simulink model "kinovaMicoSimscapeModel"  (R2021b)
settings: Solver=VariableStepAuto  StartTime=0.0  StopTime=0.3  FixedStep=0.01  RelTol=1e-3
PostLoadFcn:
  | micoRigidBodyTreeCreation;
  | IC=deg2rad([-90,180,180,0,0,0]);
  | interactiveHomePosition=deg2rad([-90 90 177.5 90 0 0]');
  | load("./KinovaMicoSimscapeVariantConfigurations.mat");
values from neighbouring files (symbols this model uses):
  micoCandlePosition = deg2rad([0,180,180,0,0,0])    [KinovaMicoSimscapeInitializeScript.m]    (also in generatingRandomTrajectory.m)
  ViaPointsTaskSpace = [ViaPointsTaskSpace;[[pi;0;pi],[pi;0;pi],[pi;0;pi],[pi;0;pi],[0;0;0],[0;0;0],[pi;0;pi]]]    [KinovaMicoSimscapeInitializeScript.m]    (also in generatingRandomTrajectory.m = [ViaPointsTaskSpace;zeros(3,7)])
undefined symbols (not defined in the file or in its folder): Mico, ViaPointsJointSpace, X, Y, Z
libraries: sm_lib x26, nesl_utility x19, robotcorelib x4, robotmaniplib x3, pid_lib x2
(part 7 of 50)

== matlab function kinovaMicoSimscapeModel/Variant Subsystem/JointSpaceController/HybridImpedanceVelocityControl/C_RNE_SKEWSYMETRIC ==
  data: q input; C output; dq input
function C = fcn(q,dq)

%% Defining the position and velocity joint variables
q1 = q(1);
q2 = q(2);
q3 = q(3);
q4 = q(4);
q5 = q(5);
q6 = q(6);

dq1 = dq(1);
dq2 = dq(2);
dq3 = dq(3);
dq4 = dq(4);
dq5 = dq(5);
dq6 = dq(6);

%% Defining each entry in the matrix

C1_1 = 0.0009968*sin(q3 - 2.0*q2 + q4 + q5)*(dq3 - 2.0*dq2 + dq4 + dq5) - 0.0009968*sin(q3 + q4 + q5)*(dq3 + dq4 + dq5) + 0.0042912*sin(q3 + q4)*(dq3 + dq4) + 0.001151*sin(q3 + q5)*(dq3 + dq5) - 0.000096245*sin(q4 + q5)*(dq4 + dq5) + 0.074028*dq2*sin(2.0*q2) - 0.0010525*dq4*sin(2.0*q4) + 0.00016499*dq5*sin(2.0*q5) - 0.0042912*sin(q3 - 2.0*q2 + q4)*(dq3 - 2.0*dq2 + dq4) - 0.001151*sin(q3 - 2.0*q2 + q5)*(dq3 - 2.0*dq2 + dq5) + 0.00033227*sin(q3 + q4 - 1.0*q5)*(dq3 + dq4 - 1.0*dq5) - 0.00033227*sin(q3 - 1.0*q4 + q5)*(dq3 - 1.0*dq4 + dq5) + 0.0009968*sin(q4 - 1.0*q3 + q5)*(dq4 - 1.0*dq3 + dq5) - 0.0009968*sin(2.0*q2 - 1.0*q3 + q4 + q5)*(2.0*dq2 - 1.0*dq3 + dq4 + dq5) - 0.00057005*sin(2.0*q3 - 2.0*q2 + q4 + q5)*(2.0*dq3 - 2.0*dq2 + dq4 + dq5) + 0.00057005*sin(2.0*q2 - 2.0*q3 + q4 + q5)*(2.0*dq2 - 2.0*dq3 + dq4 + dq5) - 0.0042912*sin(q3 - 1.0*q4)*(dq3 - 1.0*dq4) + 0.001151*sin(q3 - 1.0*q5)*(dq3 - 1.0*dq5) + 0.000032082*sin(q4 - 1.0*q5)*(dq4 - 1.0*dq5) + 0.00009067*sin(2.0*q4 + q5)*(2.0*dq4 + dq5) + 0.0042912*sin(2.0*q2 - 1.0*q3 + q4)*(2.0*dq2 - 1.0*dq3 + dq4) + 0.0025555*sin(2.0*q3 - 2.0*q2 + q4)*(2.0*dq3 - 2.0*dq2 + dq4) - 0.001151*sin(2.0*q2 - 1.0*q3 + q5)*(2.0*dq2 - 1.0*dq3 + dq5) - 0.0025555*sin(2.0*q2 - 2.0*q3 + q4)*(2.0*dq2 - 2.0*dq3 + dq4) + 0.0007489*sin(2.0*q3 - 2.0*q2 + q5)*(2.0*dq3 - 2.0*dq2 + dq5) + 0.0007489*sin(2.0*q2 - 2.0*q3 + q5)*(2.0*dq2 - 2.0*dq3 + dq5) + 0.00033227*sin(2.0*q2 - 1.0*q3 + q4 - 1.0*q5)*(2.0*dq2 - 1.0*dq3 + dq4 - 1.0*dq5) - 0.00033227*sin(2.0*q2 - 1.0*q3 - 1.0*q4 + q5)*(2.0*dq2 - 1.0*dq3 - 1.0*dq4 + dq5) - 0.00025981*sin(2.0*q2 - 2.0*q3 + q4 - 1.0*q5)*(2.0*dq2 - 2.0*dq3 + dq4 - 1.0*dq5) + 0.00025981*sin(2.0*q2 - 2.0*q3 - 1.0*q4 + q5)*(2.0*dq2 - 2.0*dq3 - 1.0*dq4 + dq5) - 0.00014289*sin(2.0*q3 - 2.0*q2 + q4 + 2.0*q5)*(2.0*dq3 - 2.0*dq2 + dq4 + 2.0*dq5) - 0.000045334*sin(2.0*q3 - 2.0*q2 + 2.0*q4 + q5)*(2.0*dq3 - 2.0*dq2 + 2.0*dq4 + dq5) - 0.000047629*sin(2.0*q2 - 2.0*q3 + q4 - 2.0*q5)*(2.0*dq2 - 2.0*dq3 + dq4 - 2.0*dq5) + 0.00014289*sin(2.0*q2 - 2.0*q3 + q4 + 2.0*q5)*(2.0*dq2 - 2.0*dq3 + dq4 + 2.0*dq5) + 0.000015111*sin(2.0*q2 - 2.0*q3 - 2.0*q4 + q5)*(2.0*dq2 - 2.0*dq3 - 2.0*dq4 + dq5) - 0.000045334*sin(2.0*q2 - 2.0*q3 + 2.0*q4 + q5)*(2.0*dq2 - 2.0*dq3 + 2.0*dq4 + dq5) + 0.030397*dq3*sin(q3) + 0.00041432*dq4*sin(q4) - 0.001256*dq5*sin(q5) - 0.030397*sin(2.0*q2 - 1.0*q3)*(2.0*dq2 - 1.0*dq3) + 0.009146*sin(2.0*q2 - 2.0*q3)*(2.0*dq2 - 2.0*dq3) - 0.000030222*sin(2.0*q4 - 1.0*q5)*(2.0*dq4 - 1.0*dq5) - 0.000013749*sin(2.0*q4 - 2.0*q5)*(2.0*dq4 - 2.0*dq5) - 0.00012375*sin(2.0*q4 + 2.0*q5)*(2.0*dq4 + 2.0*dq5) + 0.00026314*sin(2.0*q3 - 2.0*q2 + 2.0*q4)*(2.0*dq3 - 2.0*dq2 + 2.0*dq4) + 0.00026314*sin(2.0*q2 - 2.0*q3 + 2.0*q4)*(2.0*dq2 - 2.0*dq3 + 2.0*dq4) + 0.00012375*sin(2.0*q3 - 2.0*q2 + 2.0*q5)*(2.0*dq3 - 2.0*dq2 + 2.0*dq5) + 0.00012375*sin(2.0*q2 - 2.0*q3 + 2.0*q5)*(2.0*dq2 - 2.0*dq3 + 2.0*dq5) + 0.000047629*sin(2.0*q2 - 2.0*q3 - 1.0*q4 + 2.0*q5)*(2.0*dq2 - 2.0*dq3 - 1.0*dq4 + 2.0*dq5) + 0.000015111*sin(2.0*q2 - 2.0*q3 + 2.0*q4 - 1.0*q5)*(2.0*dq2 - 2.0*dq3 + 2.0*dq4 - 1.0*dq5) + 0.00006187*sin(2.0*q3 - 2.0*q2 + 2.0*q4 + 2.0*q5)*(2.0*dq3 - 2.0*dq2 + 2.0*dq4 + 2.0*dq5) + 6.8745e-6*sin(2.0*q2 - 2.0*q3 - 2.0*q4 + 2.0*q5)*(2.0*dq2 - 2.0*dq3 - 2.0*dq4 + 2.0*dq5) + 6.8745e-6*sin(2.0*q2 - 2.0*q3 + 2.0*q4 - 2.0*q5)*(2.0*dq2 - 2.0*dq3 + 2.0*dq4 - 2.0*dq5) + 0.00006187*sin(2.0*q2 - 2.0*q3 + 2.0*q4 + 2.0*q5)*(2.0*dq2 - 2.0*dq3 + 2.0*dq4 + 2.0*dq5);
 
C1_2 = 0.074028*dq1*sin(2.0*q2) + 0.0034131*dq2*sin(q2) + 0.060795*dq1*cos(2.0*q2)*sin(q3) - 0.060795*dq1*sin(2.0*q2)*cos(q3) + 0.0010437*dq2*cos(q2)*sin(q3) - 0.0010437*dq2*cos(q3)*sin(q2) - 0.017165*dq2*cos(q4)*sin(q2) - 0.0010437*dq3*cos(q2)*sin(q3) + 0.0010437*dq3*cos(q3)*sin(q2) + 0.0034398*dq4*cos(q2)*sin(q3) - 0.0034398*dq4*cos(q3)*sin(q2) + 0.0006317*dq5*cos(q2)*sin(q3) - 0.0006317*dq5*cos(q3)*sin(q2) + 0.000078*dq6*cos(q2)*sin(q3) - 0.000078*dq6*cos(q3)*sin(q2) - 0.018292*dq1*cos(2.0*q2)*sin(2.0*q3) + 0.018292*dq1*cos(2.0*q3)*sin(2.0*q2) + 0.017165*dq1*sin(2.0*q2)*sin(q3)*sin(q4) - 0.002105*dq2*sin(2.0*q4)*sin(q2)*sin(q3) + 0.002105*dq3*sin(2.0*q4)*sin(q2)*sin(q3) - 0.0010525*dq1*cos(2.0*q2)*cos(2.0*q4)*sin(2.0*q3) + 0.0010525*dq1*cos(2.0*q3)*cos(2.0*q4)*sin(2.0*q2) - 0.00049498*dq1*cos(2.0*q2)*cos(2.0*q5)*sin(2.0*q3) + 0.00049498*dq1*cos(2.0*q3)*cos(2.0*q5)*sin(2.0*q2) + 0.0004144*dq2*cos(q2)*cos(q3)*sin(q4) - 0.010222*dq2*cos(q2)*cos(q4)*sin(q3) + 0.010222*dq2*cos(q3)*cos(q4)*sin(q2) + 0.00011113*dq2*cos(q2)*cos(q5)*sin(q3) - 0.00011113*dq2*cos(q3)*cos(q5)*sin(q2) - 0.0004144*dq3*cos(q2)*cos(q3)*sin(q4) + 0.010222*dq3*cos(q2)*cos(q4)*sin(q3) - 0.010222*dq3*cos(q3)*cos(q4)*sin(q2) + 0.0026581*dq2*cos(q4)*cos(q5)*sin(q2) - 0.00011113*dq3*cos(q2)*cos(q5)*sin(q3) + 0.00011113*dq3*cos(q3)*cos(q5)*sin(q2) - 0.0004144*dq4*cos(q2)*cos(q4)*sin(q3) + 0.0004144*dq4*cos(q3)*cos(q4)*sin(q2) - 0.00024178*dq4*cos(q2)*cos(q5)*sin(q3) + 0.00024178*dq4*cos(q3)*cos(q5)*sin(q2) + 0.0010941*dq5*cos(q2)*cos(q3)*sin(q4) - 0.00011114*dq5*cos(q2)*cos(q3)*sin(q5) - 0.00024178*dq5*cos(q2)*cos(q5)*sin(q3) + 0.00024178*dq5*cos(q3)*cos(q5)*sin(q2) + 0.0001351*dq6*cos(q2)*cos(q3)*sin(q4) + 0.000234*dq6*cos(q2)*cos(q5)*sin(q3) - 0.000234*dq6*cos(q3)*cos(q5)*sin(q2) + 0.0004144*dq2*sin(q2)*sin(q3)*sin(q4) - 0.0004144*dq3*sin(q2)*sin(q3)*sin(q4) - 0.0053163*dq2*sin(q2)*sin(q4)*sin(q5) + 0.0010941*dq5*sin(q2)*sin(q3)*sin(q4) - 0.00011114*dq5*sin(q2)*sin(q3)*sin(q5) + 0.0001351*dq6*sin(q2)*sin(q3)*sin(q4) - 0.010222*dq1*cos(2.0*q2)*cos(2.0*q3)*sin(q4) - 0.0029956*dq1*cos(2.0*q2)*sin(2.0*q3)*cos(q5) + 0.0029956*dq1*cos(2.0*q3)*sin(2.0*q2)*cos(q5) - 0.010222*dq1*sin(2.0*q2)*sin(2.0*q3)*sin(q4) + 0.017165*dq1*cos(2.0*q2)*cos(q3)*sin(q4) + 0.004604*dq1*cos(2.0*q2)*cos(q5)*sin(q3) - 0.004604*dq1*sin(2.0*q2)*cos(q3)*cos(q5) - 0.002105*dq2*sin(2.0*q4)*cos(q2)*cos(q3) + 0.002105*dq3*sin(2.0*q4)*cos(q2)*cos(q3) + 0.002105*dq4*cos(2.0*q4)*cos(q2)*sin(q3) - 0.002105*dq4*cos(2.0*q4)*cos(q3)*sin(q2) - 0.00032998*dq4*cos(2.0*q5)*cos(q2)*sin(q3) + 0.00032998*dq4*cos(2.0*q5)*cos(q3)*sin(q2) + 0.00038102*dq1*cos(2.0*q2)*cos(2.0*q3)*cos(2.0*q5)*sin(q4) + 0.00076206*dq1*cos(2.0*q2)*cos(2.0*q3)*sin(2.0*q5)*cos(q4) + 0.00012089*dq1*cos(2.0*q2)*cos(2.0*q4)*sin(2.0*q3)*cos(q5) - 0.00012089*dq1*cos(2.0*q3)*cos(2.0*q4)*sin(2.0*q2)*cos(q5) - 0.00024178*dq1*cos(2.0*q2)*sin(2.0*q3)*sin(2.0*q4)*sin(q5) + 0.00024178*dq1*cos(2.0*q3)*sin(2.0*q2)*sin(2.0*q4)*sin(q5) + 0.00038102*dq1*cos(2.0*q5)*sin(2.0*q2)*sin(2.0*q3)*sin(q4) + 0.00076206*dq1*sin(2.0*q2)*sin(2.0*q3)*sin(2.0*q5)*cos(q4) - 0.00012839*dq2*cos(q2)*cos(q3)*cos(q4)*sin(q5) - 0.00006421*dq2*cos(q2)*cos(q3)*cos(q5)*sin(q4) + 0.0012409*dq2*cos(q2)*cos(q4)*cos(q5)*sin(q3) - 0.0012409*dq2*cos(q3)*cos(q4)*cos(q5)*sin(q2) + 0.00012839*dq3*cos(q2)*cos(q3)*cos(q4)*sin(q5) + 0.00006421*dq3*cos(q2)*cos(q3)*cos(q5)*sin(q4) - 0.0012409*dq3*cos(q2)*cos(q4)*cos(q5)*sin(q3) + 0.0012409*dq3*cos(q3)*cos(q4)*cos(q5)*sin(q2) + 0.00006421*dq4*cos(q2)*cos(q4)*cos(q5)*sin(q3) - 0.00006421*dq4*cos(q3)*cos(q4)*cos(q5)*sin(q2) + 0.00041878*dq5*cos(q2)*cos(q3)*cos(q4)*sin(q5) + 1.5e-8*dq5*cos(q2)*cos(q3)*cos(q5)*sin(q4) + 0.00012839*dq5*cos(q2)*cos(q4)*cos(q5)*sin(q3) - 0.00012839*dq5*cos(q3)*cos(q4)*cos(q5)*sin(q2) - 0.0002702*dq6*cos(q2)*cos(q3)*cos(q4)*sin(q5) - 0.0001351*dq6*cos(q2)*cos(q3)*cos(q5)*sin(q4) - 0.0033193*dq2*cos(q2)*sin(q3)*sin(q4)*sin(q5) + 0.0033193*dq2*cos(q3)*sin(q2)*sin(q4)*sin(q5) - 0.00012839*dq2*cos(q4)*sin(q2)*sin(q3)*sin(q5) - 0.00006421*dq2*cos(q5)*sin(q2)*sin(q3)*sin(q4) + 0.0033193*dq3*cos(q2)*sin(q3)*sin(q4)*sin(q5) - 0.0033193*dq3*cos(q3)*sin(q2)*sin(q4)*sin(q5) + 0.00012839*dq3*cos(q4)*sin(q2)*sin(q3)*sin(q5) + 0.00006421*dq3*cos(q5)*sin(q2)*sin(q3)*sin(q4) - 0.00012839*dq4*cos(q2)*sin(q3)*sin(q4)*sin(q5) + 0.00012839*dq4*cos(q3)*sin(q2)*sin(q4)*sin(q5) - 0.000064215*dq5*cos(q2)*sin(q3)*sin(q4)*sin(q5) + 0.000064215*dq5*cos(q3)*sin(q2)*sin(q4)*sin(q5) + 0.00041878*dq5*cos(q4)*sin(q2)*sin(q3)*sin(q5) + 1.5e-8*dq5*cos(q5)*sin(q2)*sin(q3)*sin(q4) - 0.0002702*dq6*cos(q4)*sin(q2)*sin(q3)*sin(q5) - 0.0001351*dq6*cos(q5)*sin(q2)*sin(q3)*sin(q4) + 0.0033194*dq1*cos(2.0*q2)*cos(2.0*q3)*cos(q4)*sin(q5) + 0.001241*dq1*cos(2.0*q2)*cos(2.0*q3)*cos(q5)*sin(q4) - 0.00043998*dq2*cos(2.0*q4)*sin(2.0*q5)*cos(q2)*cos(q3) - 0.00054998*dq2*cos(2.0*q5)*sin(2.0*q4)*cos(q2)*cos(q3) + 0.00043998*dq3*cos(2.0*q4)*sin(2.0*q5)*cos(q2)*cos(q3) + 0.00054998*dq3*cos(2.0*q5)*sin(2.0*q4)*cos(q2)*cos(q3) + 0.00054998*dq4*cos(2.0*q4)*cos(2.0*q5)*cos(q2)*sin(q3) - 0.00054998*dq4*cos(2.0*q4)*cos(2.0*q5)*cos(q3)*sin(q2) + 0.00043998*dq5*cos(2.0*q4)*cos(2.0*q5)*cos(q2)*sin(q3) - 0.00043998*dq5*cos(2.0*q4)*cos(2.0*q5)*cos(q3)*sin(q2) + 0.0033194*dq1*sin(2.0*q2)*sin(2.0*q3)*cos(q4)*sin(q5) + 0.001241*dq1*sin(2.0*q2)*sin(2.0*q3)*cos(q5)*sin(q4) - 0.00043998*dq2*cos(2.0*q4)*sin(2.0*q5)*sin(q2)*sin(q3) - 0.00054998*dq2*cos(2.0*q5)*sin(2.0*q4)*sin(q2)*sin(q3) + 0.00043998*dq3*cos(2.0*q4)*sin(2.0*q5)*sin(q2)*sin(q3) + 0.00054998*dq3*cos(2.0*q5)*sin(2.0*q4)*sin(q2)*sin(q3) - 0.00043998*dq4*sin(2.0*q4)*sin(2.0*q5)*cos(q2)*sin(q3) + 0.00043998*dq4*sin(2.0*q4)*sin(2.0*q5)*cos(q3)*sin(q2) - 0.00054998*dq5*sin(2.0*q4)*sin(2.0*q5)*cos(q2)*sin(q3) + 0.00054998*dq5*sin(2.0*q4)*sin(2.0*q5)*cos(q3)*sin(q2) - 0.00027498*dq1*cos(2.0*q2)*cos(2.0*q4)*cos(2.0*q5)*sin(2.0*q3) + 0.00027498*dq1*cos(2.0*q3)*cos(2.0*q4)*cos(2.0*q5)*sin(2.0*q2) + 0.00021998*dq1*cos(2.0*q2)*sin(2.0*q3)*sin(2.0*q4)*sin(2.0*q5) - 0.00021998*dq1*cos(2.0*q3)*sin(2.0*q2)*sin(2.0*q4)*sin(2.0*q5) - 0.0053163*dq1*cos(2.0*q2)*cos(q3)*cos(q4)*sin(q5) - 0.0026581*dq1*cos(2.0*q2)*cos(q3)*cos(q5)*sin(q4) + 0.00048357*dq2*cos(2.0*q4)*cos(q2)*cos(q3)*sin(q5) + 0.00038102*dq2*cos(2.0*q5)*cos(q2)*cos(q4)*sin(q3) - 0.00038102*dq2*cos(2.0*q5)*cos(q3)*cos(q4)*sin(q2) + 0.00024179*dq2*sin(2.0*q4)*cos(q2)*cos(q3)*cos(q5) - 0.00048357*dq3*cos(2.0*q4)*cos(q2)*cos(q3)*sin(q5) - 0.00038102*dq3*cos(2.0*q5)*cos(q2)*cos(q4)*sin(q3) + 0.00038102*dq3*cos(2.0*q5)*cos(q3)*cos(q4)*sin(q2) - 0.00024179*dq3*sin(2.0*q4)*cos(q2)*cos(q3)*cos(q5) - 0.00024179*dq4*cos(2.0*q4)*cos(q2)*cos(q5)*sin(q3) + 0.00024179*dq4*cos(2.0*q4)*cos(q3)*cos(q5)*sin(q2) - 0.00024178*dq5*cos(2.0*q4)*cos(q2)*cos(q5)*sin(q3) + 0.00024178*dq5*cos(2.0*q4)*cos(q3)*cos(q5)*sin(q2) - 0.00076206*dq5*cos(2.0*q5)*cos(q2)*cos(q3)*sin(q4) - 0.00038102*dq5*sin(2.0*q5)*cos(q2)*cos(q3)*cos(q4) - 0.0053163*dq1*sin(2.0*q2)*cos(q4)*sin(q3)*sin(q5) - 0.0026581*dq1*sin(2.0*q2)*cos(q5)*sin(q3)*sin(q4) + 0.00048357*dq2*cos(2.0*q4)*sin(q2)*sin(q3)*sin(q5) + 0.00024179*dq2*sin(2.0*q4)*cos(q5)*sin(q2)*sin(q3) - 0.00076206*dq2*sin(2.0*q5)*cos(q2)*sin(q3)*sin(q4) + 0.00076206*dq2*sin(2.0*q5)*cos(q3)*sin(q2)*sin(q4) - 0.00048357*dq3*cos(2.0*q4)*sin(q2)*sin(q3)*sin(q5) - 0.00024179*dq3*sin(2.0*q4)*cos(q5)*sin(q2)*sin(q3) + 0.00076206*dq3*sin(2.0*q5)*cos(q2)*sin(q3)*sin(q4) - 0.00076206*dq3*sin(2.0*q5)*cos(q3)*sin(q2)*sin(q4) + 0.00048357*dq4*sin(2.0*q4)*cos(q2)*sin(q3)*sin(q5) - 0.00048357*dq4*sin(2.0*q4)*cos(q3)*sin(q2)*sin(q5) - 0.00076206*dq5*cos(2.0*q5)*sin(q2)*sin(q3)*sin(q4) + 0.00012089*dq5*sin(2.0*q4)*cos(q2)*sin(q3)*sin(q5) - 0.00012089*dq5*sin(2.0*q4)*cos(q3)*sin(q2)*sin(q5) - 0.00038102*dq5*sin(2.0*q5)*cos(q4)*sin(q2)*sin(q3);
 
C1_3 = 0.030397*dq1*sin(q3) - 0.030397*dq1*cos(2.0*q2)*sin(q3) + 0.030397*dq1*sin(2.0*q2)*cos(q3) - 0.0010437*dq2*cos(q2)*sin(q3) + 0.0010437*dq2*cos(q3)*sin(q2) + 0.0085823*dq1*cos(q3)*sin(q4) + 0.0010437*dq3*cos(q2)*sin(q3) - 0.0010437*dq3*cos(q3)*sin(q2) + 0.002302*dq1*cos(q5)*sin(q3) - 0.0034398*dq4*cos(q2)*sin(q3) + 0.0034398*dq4*cos(q3)*sin(q2) - 0.0006317*dq5*cos(q2)*sin(q3) + 0.0006317*dq5*cos(q3)*sin(q2) - 0.000078*dq6*cos(q2)*sin(q3) + 0.000078*dq6*cos(q3)*sin(q2) + 0.018292*dq1*cos(2.0*q2)*sin(2.0*q3) - 0.018292*dq1*cos(2.0*q3)*sin(2.0*q2) - 0.0085823*dq1*sin(2.0*q2)*sin(q3)*sin(q4) + 0.002105*dq2*sin(2.0*q4)*sin(q2)*sin(q3) - 0.002105*dq3*sin(2.0*q4)*sin(q2)*sin(q3) + 0.0010525*dq1*cos(2.0*q2)*cos(2.0*q4)*sin(2.0*q3) - 0.0010525*dq1*cos(2.0*q3)*cos(2.0*q4)*sin(2.0*q2) + 0.00049498*dq1*cos(2.0*q2)*cos(2.0*q5)*sin(2.0*q3) - 0.00049498*dq1*cos(2.0*q3)*cos(2.0*q5)*sin(2.0*q2) - 0.0004144*dq2*cos(q2)*cos(q3)*sin(q4) + 0.010222*dq2*cos(q2)*cos(q4)*sin(q3) - 0.010222*dq2*cos(q3)*cos(q4)*sin(q2) - 0.00011113*dq2*cos(q2)*cos(q5)*sin(q3) + 0.00011113*dq2*cos(q3)*cos(q5)*sin(q2) + 0.0004144*dq3*cos(q2)*cos(q3)*sin(q4) - 0.010222*dq3*cos(q2)*cos(q4)*sin(q3) + 0.010222*dq3*cos(q3)*cos(q4)*sin(q2) - 0.0026581*dq1*cos(q3)*cos(q4)*sin(q5) - 0.0013291*dq1*cos(q3)*cos(q5)*sin(q4) + 0.00011113*dq3*cos(q2)*cos(q5)*sin(q3) - 0.00011113*dq3*cos(q3)*cos(q5)*sin(q2) + 0.0004144*dq4*cos(q2)*cos(q4)*sin(q3) - 0.0004144*dq4*cos(q3)*cos(q4)*sin(q2) + 0.00024178*dq4*cos(q2)*cos(q5)*sin(q3) - 0.00024178*dq4*cos(q3)*cos(q5)*sin(q2) - 0.0010941*dq5*cos(q2)*cos(q3)*sin(q4) + 0.00011114*dq5*cos(q2)*cos(q3)*sin(q5) + 0.00024178*dq5*cos(q2)*cos(q5)*sin(q3) - 0.00024178*dq5*cos(q3)*cos(q5)*sin(q2) - 0.0001351*dq6*cos(q2)*cos(q3)*sin(q4) - 0.000234*dq6*cos(q2)*cos(q5)*sin(q3) + 0.000234*dq6*cos(q3)*cos(q5)*sin(q2) - 0.0004144*dq2*sin(q2)*sin(q3)*sin(q4) + 0.0004144*dq3*sin(q2)*sin(q3)*sin(q4) - 0.0010941*dq5*sin(q2)*sin(q3)*sin(q4) + 0.00011114*dq5*sin(q2)*sin(q3)*sin(q5) - 0.0001351*dq6*sin(q2)*sin(q3)*sin(q4) + 0.010222*dq1*cos(2.0*q2)*cos(2.0*q3)*sin(q4) + 0.0029956*dq1*cos(2.0*q2)*sin(2.0*q3)*cos(q5) - 0.0029956*dq1*cos(2.0*q3)*sin(2.0*q2)*cos(q5) + 0.010222*dq1*sin(2.0*q2)*sin(2.0*q3)*sin(q4) - 0.0085823*dq1*cos(2.0*q2)*cos(q3)*sin(q4) - 0.002302*dq1*cos(2.0*q2)*cos(q5)*sin(q3) + 0.002302*dq1*sin(2.0*q2)*cos(q3)*cos(q5) + 0.002105*dq2*sin(2.0*q4)*cos(q2)*cos(q3) - 0.002105*dq3*sin(2.0*q4)*cos(q2)*cos(q3) - 0.002105*dq4*cos(2.0*q4)*cos(q2)*sin(q3) + 0.002105*dq4*cos(2.0*q4)*cos(q3)*sin(q2) + 0.00032998*dq4*cos(2.0*q5)*cos(q2)*sin(q3) - 0.00032998*dq4*cos(2.0*q5)*cos(q3)*sin(q2) - 0.00038102*dq1*cos(2.0*q2)*cos(2.0*q3)*cos(2.0*q5)*sin(q4) - 0.00076206*dq1*cos(2.0*q2)*cos(2.0*q3)*sin(2.0*q5)*cos(q4) - 0.00012089*dq1*cos(2.0*q2)*cos(2.0*q4)*sin(2.0*q3)*cos(q5) + 0.00012089*dq1*cos(2.0*q3)*cos(2.0*q4)*sin(2.0*q2)*cos(q5) + 0.00024178*dq1*cos(2.0*q2)*sin(2.0*q3)*sin(2.0*q4)*sin(q5) - 0.00024178*dq1*cos(2.0*q3)*sin(2.0*q2)*sin(2.0*q4)*sin(q5) - 0.00038102*dq1*cos(2.0*q5)*sin(2.0*q2)*sin(2.0*q3)*sin(q4) - 0.00076206*dq1*sin(2.0*q2)*sin(2.0*q3)*sin(2.0*q5)*cos(q4) + 0.00012839*dq2*cos(q2)*cos(q3)*cos(q4)*sin(q5) + 0.00006421*dq2*cos(q2)*cos(q3)*cos(q5)*sin(q4) - 0.0012409*dq2*cos(q2)*cos(q4)*cos(q5)*sin(q3) + 0.0012409*dq2*cos(q3)*cos(q4)*cos(q5)*sin(q2) - 0.00012839*dq3*cos(q2)*cos(q3)*cos(q4)*sin(q5) - 0.00006421*dq3*cos(q2)*cos(q3)*cos(q5)*sin(q4) + 0.0012409*dq3*cos(q2)*cos(q4)*cos(q5)*sin(q3) - 0.0012409*dq3*cos(q3)*cos(q4)*cos(q5)*sin(q2) - 0.00006421*dq4*cos(q2)*cos(q4)*cos(q5)*sin(q3) + 0.00006421*dq4*cos(q3)*cos(q4)*cos(q5)*sin(q2) - 0.00041878*dq5*cos(q2)*cos(q3)*cos(q4)*sin(q5) - 1.5e-8*dq5*cos(q2)*cos(q3)*cos(q5)*sin(q4) - 0.00012839*dq5*cos(q2)*cos(q4)*cos(q5)*sin(q3) + 0.00012839*dq5*cos(q3)*cos(q4)*cos(q5)*sin(q2) + 0.0002702*dq6*cos(q2)*cos(q3)*cos(q4)*sin(q5) + 0.0001351*dq6*cos(q2)*cos(q3)*cos(q5)*sin(q4) + 0.0033193*dq2*cos(q2)*sin(q3)*sin(q4)*sin(q5) - 0.0033193*dq2*cos(q3)*sin(q2)*sin(q4)*sin(q5) + 0.00012839*dq2*cos(q4)*sin(q2)*sin(q3)*sin(q5) + 0.00006421*dq2*cos(q5)*sin(q2)*sin(q3)*sin(q4) - 0.0033193*dq3*cos(q2)*sin(q3)*sin(q4)*sin(q5) + 0.0033193*dq3*cos(q3)*sin(q2)*sin(q4)*sin(q5) - 0.00012839*dq3*cos(q4)*sin(q2)*sin(q3)*sin(q5) - 0.00006421*dq3*cos(q5)*sin(q2)*sin(q3)*sin(q4) + 0.00012839*dq4*cos(q2)*sin(q3)*sin(q4)*sin(q5) - 0.00012839*dq4*cos(q3)*sin(q2)*sin(q4)*sin(q5) + 0.000064215*dq5*cos(q2)*sin(q3)*sin(q4)*sin(q5) - 0.000064215*dq5*cos(q3)*sin(q2)*sin(q4)*sin(q5) - 0.00041878*dq5*cos(q4)*sin(q2)*sin(q3)*sin(q5) - 1.5e-8*dq5*cos(q5)*sin(q2)*sin(q3)*sin(q4) + 0.0002702*dq6*cos(q4)*sin(q2)*sin(q3)*sin(q5) + 0.0001351*dq6*cos(q5)*sin(q2)*sin(q3)*sin(q4) - 0.0033194*dq1*cos(2.0*q2)*cos(2.0*q3)*cos(q4)*sin(q5) - 0.001241*dq1*cos(2.0*q2)*cos(2.0*q3)*cos(q5)*sin(q4) + 0.00043998*dq2*cos(2.0*q4)*sin(2.0*q5)*cos(q2)*cos(q3) + 0.00054998*dq2*cos(2.0*q5)*sin(2.0*q4)*cos(q2)*cos(q3) - 0.00043998*dq3*cos(2.0*q4)*sin(2.0*q5)*cos(q2)*cos(q3) - 0.00054998*dq3*cos(2.0*q5)*sin(2.0*q4)*cos(q2)*cos(q3) - 0.00054998*dq4*cos(2.0*q4)*cos(2.0*q5)*cos(q2)*sin(q3) + 0.00054998*dq4*cos(2.0*q4)*cos(2.0*q5)*cos(q3)*sin(q2) - 0.00043998*dq5*cos(2.0*q4)*cos(2.0*q5)*cos(q2)*sin(q3) + 0.00043998*dq5*cos(2.0*q4)*cos(2.0*q5)*cos(q3)*sin(q2) - 0.0033194*dq1*sin(2.0*q2)*sin(2.0*q3)*cos(q4)*sin(q5) - 0.001241*dq1*sin(2.0*q2)*sin(2.0*q3)*cos(q5)*sin(q4) + 0.00043998*dq2*cos(2.0*q4)*sin(2.0*q5)*sin(q2)*sin(q3) + 0.00054998*dq2*cos(2.0*q5)*sin(2.0*q4)*sin(q2)*sin(q3) - 0.00043998*dq3*cos(2.0*q4)*sin(2.0*q5)*sin(q2)*sin(q3) - 0.00054998*dq3*cos(2.0*q5)*sin(2.0*q4)*sin(q2)*sin(q3) + 0.00043998*dq4*sin(2.0*q4)*sin(2.0*q5)*cos(q2)*sin(q3) - 0.00043998*dq4*sin(2.0*q4)*sin(2.0*q5)*cos(q3)*sin(q2) + 0.00054998*dq5*sin(2.0*q4)*sin(2.0*q5)*cos(q2)*sin(q3) - 0.00054998*dq5*sin(2.0*q4)*sin(2.0*q5)*cos(q3)*sin(q2) + 0.00027498*dq1*cos(2.0*q2)*cos(2.0*q4)*cos(2.0*q5)*sin(2.0*q3) - 0.00027498*dq1*cos(2.0*q3)*cos(2.0*q4)*cos(2.0*q5)*sin(2.0*q2) - 0.00021998*dq1*cos(2.0*q2)*sin(2.0*q3)*sin(2.0*q4)*sin(2.0*q5) + 0.00021998*dq1*cos(2.0*q3)*sin(2.0*q2)*sin(2.0*q4)*sin(2.0*q5) + 0.0026581*dq1*cos(2.0*q2)*cos(q3)*cos(q4)*sin(q5) + 0.0013291*dq1*cos(2.0*q2)*cos(q3)*cos(q5)*sin(q4) - 0.00048357*dq2*cos(2.0*q4)*cos(q2)*cos(q3)*sin(q5) - 0.00038102*dq2*cos(2.0*q5)*cos(q2)*cos(q4)*sin(q3) + 0.00038102*dq2*cos(2.0*q5)*cos(q3)*cos(q4)*sin(q2) - 0.00024179*dq2*sin(2.0*q4)*cos(q2)*cos(q3)*cos(q5) + 0.00048357*dq3*cos(2.0*q4)*cos(q2)*cos(q3)*sin(q5) + 0.00038102*dq3*cos(2.0*q5)*cos(q2)*cos(q4)*sin(q3) - 0.00038102*dq3*cos(2.0*q5)*cos(q3)*cos(q4)*sin(q2) + 0.00024179*dq3*sin(2.0*q4)*cos(q2)*cos(q3)*cos(q5) + 0.00024179*dq4*cos(2.0*q4)*cos(q2)*cos(q5)*sin(q3) - 0.00024179*dq4*cos(2.0*q4)*cos(q3)*cos(q5)*sin(q2) + 0.00024178*dq5*cos(2.0*q4)*cos(q2)*cos(q5)*sin(q3) - 0.00024178*dq5*cos(2.0*q4)*cos(q3)*cos(q5)*sin(q2) + 0.00076206*dq5*cos(2.0*q5)*cos(q2)*cos(q3)*sin(q4) + 0.00038102*dq5*sin(2.0*q5)*cos(q2)*cos(q3)*cos(q4) + 0.0026581*dq1*sin(2.0*q2)*cos(q4)*sin(q3)*sin(q5) + 0.0013291*dq1*sin(2.0*q2)*cos(q5)*sin(q3)*sin(q4) - 0.00048357*dq2*cos(2.0*q4)*sin(q2)*sin(q3)*sin(q5) - 0.00024179*dq2*sin(2.0*q4)*cos(q5)*sin(q2)*sin(q3) + 0.00076206*dq2*sin(2.0*q5)*cos(q2)*sin(q3)*sin(q4) - 0.00076206*dq2*sin(2.0*q5)*cos(q3)*sin(q2)*sin(q4) + 0.00048357*dq3*cos(2.0*q4)*sin(q2)*sin(q3)*sin(q5) + 0.00024179*dq3*sin(2.0*q4)*cos(q5)*sin(q2)*sin(q3) - 0.00076206*dq3*sin(2.0*q5)*cos(q2)*sin(q3)*sin(q4) + 0.00076206*dq3*sin(2.0*q5)*cos(q3)*sin(q2)*sin(q4) - 0.00048357*dq4*sin(2.0*q4)*cos(q2)*sin(q3)*sin(q5) + 0.00048357*dq4*sin(2.0*q4)*cos(q3)*sin(q2)*sin(q5) + 0.00076206*dq5*cos(2.0*q5)*sin(q2)*sin(q3)*sin(q4) - 0.00012089*dq5*sin(2.0*q4)*cos(q2)*sin(q3)*sin(q5) + 0.00012089*dq5*sin(2.0*q4)*cos(q3)*sin(q2)*sin(q5) + 0.00038102*dq5*sin(2.0*q5)*cos(q4)*sin(q2)*sin(q3);
 
C1_4 = 0.00041432*dq1*sin(q4) - 0.0010525*dq1*sin(2.0*q4) + 0.00024178*dq1*cos(2.0*q4)*sin(q5) + 0.00012089*dq1*sin(2.0*q4)*cos(q5) + 0.0034398*dq2*cos(q2)*sin(q3) - 0.0034398*dq2*cos(q3)*sin(q2) + 0.0085823*dq1*cos(q4)*sin(q3) - 0.0034398*dq3*cos(q2)*sin(q3) + 0.0034398*dq3*cos(q3)*sin(q2) - 0.00012833*dq1*cos(q4)*sin(q5) - 0.000064164*dq1*cos(q5)*sin(q4) + 0.017165*dq4*cos(q4)*sin(q2) - 0.00021999*dq1*cos(2.0*q4)*sin(2.0*q5) - 0.00027499*dq1*cos(2.0*q5)*sin(2.0*q4) + 0.00065996*dq5*sin(2.0*q5)*sin(q2)*sin(q3) + 0.0010525*dq1*cos(2.0*q2)*cos(2.0*q3)*sin(2.0*q4) + 0.0010525*dq1*sin(2.0*q2)*sin(2.0*q3)*sin(2.0*q4) - 0.0004144*dq2*cos(q2)*cos(q4)*sin(q3) + 0.0004144*dq2*cos(q3)*cos(q4)*sin(q2) - 0.00024178*dq2*cos(q2)*cos(q5)*sin(q3) + 0.00024178*dq2*cos(q3)*cos(q5)*sin(q2) + 0.0004144*dq3*cos(q2)*cos(q4)*sin(q3) - 0.0004144*dq3*cos(q3)*cos(q4)*sin(q2) - 0.0013291*dq1*cos(q4)*cos(q5)*sin(q3) + 0.00024178*dq3*cos(q2)*cos(q5)*sin(q3) - 0.00024178*dq3*cos(q3)*cos(q5)*sin(q2) + 0.0004144*dq4*cos(q2)*cos(q3)*sin(q4) + 0.010222*dq4*cos(q2)*cos(q4)*sin(q3) - 0.010222*dq4*cos(q3)*cos(q4)*sin(q2) - 0.0010941*dq5*cos(q2)*cos(q4)*sin(q3) + 0.0010941*dq5*cos(q3)*cos(q4)*sin(q2) - 0.0026581*dq4*cos(q4)*cos(q5)*sin(q2) + 0.00024178*dq5*cos(q2)*cos(q3)*sin(q5) - 0.0001351*dq6*cos(q2)*cos(q4)*sin(q3) + 0.0001351*dq6*cos(q3)*cos(q4)*sin(q2) - 0.0053163*dq5*cos(q4)*cos(q5)*sin(q2) + 0.0026581*dq1*sin(q3)*sin(q4)*sin(q5) + 0.0004144*dq4*sin(q2)*sin(q3)*sin(q4) + 0.0053163*dq4*sin(q2)*sin(q4)*sin(q5) + 0.00024178*dq5*sin(q2)*sin(q3)*sin(q5) + 0.0026581*dq5*sin(q2)*sin(q4)*sin(q5) + 0.005111*dq1*cos(2.0*q2)*sin(2.0*q3)*cos(q4) - 0.005111*dq1*cos(2.0*q3)*sin(2.0*q2)*cos(q4) - 0.0085823*dq1*cos(2.0*q2)*cos(q4)*sin(q3) + 0.0085823*dq1*sin(2.0*q2)*cos(q3)*cos(q4) + 0.002105*dq2*cos(2.0*q4)*cos(q2)*sin(q3) - 0.002105*dq2*cos(2.0*q4)*cos(q3)*sin(q2) - 0.00032998*dq2*cos(2.0*q5)*cos(q2)*sin(q3) + 0.00032998*dq2*cos(2.0*q5)*cos(q3)*sin(q2) - 0.002105*dq3*cos(2.0*q4)*cos(q2)*sin(q3) + 0.002105*dq3*cos(2.0*q4)*cos(q3)*sin(q2) + 0.00032998*dq3*cos(2.0*q5)*cos(q2)*sin(q3) - 0.00032998*dq3*cos(2.0*q5)*cos(q3)*sin(q2) + 0.00065996*dq5*sin(2.0*q5)*cos(q2)*cos(q3) - 0.00024178*dq1*cos(2.0*q2)*cos(2.0*q3)*cos(2.0*q4)*sin(q5) - 0.00012089*dq1*cos(2.0*q2)*cos(2.0*q3)*sin(2.0*q4)*cos(q5) - 0.00019051*dq1*cos(2.0*q2)*cos(2.0*q5)*sin(2.0*q3)*cos(q4) + 0.00019051*dq1*cos(2.0*q3)*cos(2.0*q5)*sin(2.0*q2)*cos(q4) + 0.00038103*dq1*cos(2.0*q2)*sin(2.0*q3)*sin(2.0*q5)*sin(q4) - 0.00038103*dq1*cos(2.0*q3)*sin(2.0*q2)*sin(2.0*q5)*sin(q4) - 0.00024178*dq1*cos(2.0*q4)*sin(2.0*q2)*sin(2.0*q3)*sin(q5) - 0.00012089*dq1*sin(2.0*q2)*sin(2.0*q3)*sin(2.0*q4)*cos(q5) + 0.00006421*dq2*cos(q2)*cos(q4)*cos(q5)*sin(q3) - 0.00006421*dq2*cos(q3)*cos(q4)*cos(q5)*sin(q2) - 0.00006421*dq3*cos(q2)*cos(q4)*cos(q5)*sin(q3) + 0.00006421*dq3*cos(q3)*cos(q4)*cos(q5)*sin(q2) - 0.00012839*dq4*cos(q2)*cos(q3)*cos(q4)*sin(q5) - 0.00006421*dq4*cos(q2)*cos(q3)*cos(q5)*sin(q4) - 0.0012409*dq4*cos(q2)*cos(q4)*cos(q5)*sin(q3) + 0.0012409*dq4*cos(q3)*cos(q4)*cos(q5)*sin(q2) - 0.000064215*dq5*cos(q2)*cos(q3)*cos(q4)*sin(q5) - 0.00012839*dq5*cos(q2)*cos(q3)*cos(q5)*sin(q4) - 0.0033193*dq5*cos(q2)*cos(q4)*cos(q5)*sin(q3) + 0.0033193*dq5*cos(q3)*cos(q4)*cos(q5)*sin(q2) + 0.0001351*dq6*cos(q2)*cos(q4)*cos(q5)*sin(q3) - 0.0001351*dq6*cos(q3)*cos(q4)*cos(q5)*sin(q2) - 0.00012839*dq2*cos(q2)*sin(q3)*sin(q4)*sin(q5) + 0.00012839*dq2*cos(q3)*sin(q2)*sin(q4)*sin(q5) + 0.00012839*dq3*cos(q2)*sin(q3)*sin(q4)*sin(q5) - 0.00012839*dq3*cos(q3)*sin(q2)*sin(q4)*sin(q5) + 0.0033193*dq4*cos(q2)*sin(q3)*sin(q4)*sin(q5) - 0.0033193*dq4*cos(q3)*sin(q2)*sin(q4)*sin(q5) - 0.00012839*dq4*cos(q4)*sin(q2)*sin(q3)*sin(q5) - 0.00006421*dq4*cos(q5)*sin(q2)*sin(q3)*sin(q4) + 0.0016597*dq5*cos(q2)*sin(q3)*sin(q4)*sin(q5) - 0.0016597*dq5*cos(q3)*sin(q2)*sin(q4)*sin(q5) - 0.000064215*dq5*cos(q4)*sin(q2)*sin(q3)*sin(q5) - 0.00012839*dq5*cos(q5)*sin(q2)*sin(q3)*sin(q4) - 0.0002702*dq6*cos(q2)*sin(q3)*sin(q4)*sin(q5) + 0.0002702*dq6*cos(q3)*sin(q2)*sin(q4)*sin(q5) - 0.00062049*dq1*cos(2.0*q2)*sin(2.0*q3)*cos(q4)*cos(q5) + 0.00062049*dq1*cos(2.0*q3)*sin(2.0*q2)*cos(q4)*cos(q5) + 0.00054998*dq2*cos(2.0*q4)*cos(2.0*q5)*cos(q2)*sin(q3) - 0.00054998*dq2*cos(2.0*q4)*cos(2.0*q5)*cos(q3)*sin(q2) - 0.00054998*dq3*cos(2.0*q4)*cos(2.0*q5)*cos(q2)*sin(q3) + 0.00054998*dq3*cos(2.0*q4)*cos(2.0*q5)*cos(q3)*sin(q2) + 0.0016597*dq1*cos(2.0*q2)*sin(2.0*q3)*sin(q4)*sin(q5) - 0.0016597*dq1*cos(2.0*q3)*sin(2.0*q2)*sin(q4)*sin(q5) - 0.00043998*dq2*sin(2.0*q4)*sin(2.0*q5)*cos(q2)*sin(q3) + 0.00043998*dq2*sin(2.0*q4)*sin(2.0*q5)*cos(q3)*sin(q2) + 0.00043998*dq3*sin(2.0*q4)*sin(2.0*q5)*cos(q2)*sin(q3) - 0.00043998*dq3*sin(2.0*q4)*sin(2.0*q5)*cos(q3)*sin(q2) + 0.00021998*dq1*cos(2.0*q2)*cos(2.0*q3)*cos(2.0*q4)*sin(2.0*q5) + 0.00027498*dq1*cos(2.0*q2)*cos(2.0*q3)*cos(2.0*q5)*sin(2.0*q4) + 0.00021998*dq1*cos(2.0*q4)*sin(2.0*q2)*sin(2.0*q3)*sin(2.0*q5) + 0.00027498*dq1*cos(2.0*q5)*sin(2.0*q2)*sin(2.0*q3)*sin(2.0*q4) + 0.0013291*dq1*cos(2.0*q2)*cos(q4)*cos(q5)*sin(q3) - 0.0013291*dq1*sin(2.0*q2)*cos(q3)*cos(q4)*cos(q5) - 0.00024179*dq2*cos(2.0*q4)*cos(q2)*cos(q5)*sin(q3) + 0.00024179*dq2*cos(2.0*q4)*cos(q3)*cos(q5)*sin(q2) + 0.00024179*dq3*cos(2.0*q4)*cos(q2)*cos(q5)*sin(q3) - 0.00024179*dq3*cos(2.0*q4)*cos(q3)*cos(q5)*sin(q2) - 0.00038102*dq4*cos(2.0*q5)*cos(q2)*cos(q4)*sin(q3) + 0.00038102*dq4*cos(2.0*q5)*cos(q3)*cos(q4)*sin(q2) - 0.00076206*dq5*cos(2.0*q5)*cos(q2)*cos(q4)*sin(q3) + 0.00076206*dq5*cos(2.0*q5)*cos(q3)*cos(q4)*sin(q2) - 0.0026581*dq1*cos(2.0*q2)*sin(q3)*sin(q4)*sin(q5) + 0.0026581*dq1*sin(2.0*q2)*cos(q3)*sin(q4)*sin(q5) + 0.00048357*dq2*sin(2.0*q4)*cos(q2)*sin(q3)*sin(q5) - 0.00048357*dq2*sin(2.0*q4)*cos(q3)*sin(q2)*sin(q5) - 0.00048357*dq3*sin(2.0*q4)*cos(q2)*sin(q3)*sin(q5) + 0.00048357*dq3*sin(2.0*q4)*cos(q3)*sin(q2)*sin(q5) + 0.00076206*dq4*sin(2.0*q5)*cos(q2)*sin(q3)*sin(q4) - 0.00076206*dq4*sin(2.0*q5)*cos(q3)*sin(q2)*sin(q4) + 0.00038102*dq5*sin(2.0*q5)*cos(q2)*sin(q3)*sin(q4) - 0.00038102*dq5*sin(2.0*q5)*cos(q3)*sin(q2)*sin(q4);
 
C1_5 = 0.00016499*dq1*sin(2.0*q5) - 0.001256*dq1*sin(q5) + 0.000060447*dq1*cos(2.0*q4)*sin(q5) + 0.00012089*dq1*sin(2.0*q4)*cos(q5) + 0.0006317*dq2*cos(q2)*sin(q3) - 0.0006317*dq2*cos(q3)*sin(q2) - 0.0006317*dq3*cos(q2)*sin(q3) + 0.0006317*dq3*cos(q3)*sin(q2) + 0.002302*dq1*cos(q3)*sin(q5) - 0.000064164*dq1*cos(q4)*sin(q5) - 0.00012833*dq1*cos(q5)*sin(q4) - 0.00027499*dq1*cos(2.0*q4)*sin(2.0*q5) - 0.00021999*dq1*cos(2.0*q5)*sin(2.0*q4) - 0.002302*dq1*sin(2.0*q2)*sin(q3)*sin(q5) + 0.00065996*dq4*sin(2.0*q5)*sin(q2)*sin(q3) + 0.00049498*dq1*cos(2.0*q2)*cos(2.0*q3)*sin(2.0*q5) + 0.00049498*dq1*sin(2.0*q2)*sin(2.0*q3)*sin(2.0*q5) + 0.0010941*dq2*cos(q2)*cos(q3)*sin(q4) - 0.00011114*dq2*cos(q2)*cos(q3)*sin(q5) - 0.00024178*dq2*cos(q2)*cos(q5)*sin(q3) + 0.00024178*dq2*cos(q3)*cos(q5)*sin(q2) - 0.0010941*dq3*cos(q2)*cos(q3)*sin(q4) - 0.0026581*dq1*cos(q4)*cos(q5)*sin(q3) + 0.00011114*dq3*cos(q2)*cos(q3)*sin(q5) + 0.00024178*dq3*cos(q2)*cos(q5)*sin(q3) - 0.00024178*dq3*cos(q3)*cos(q5)*sin(q2) - 0.0010941*dq4*cos(q2)*cos(q4)*sin(q3) + 0.0010941*dq4*cos(q3)*cos(q4)*sin(q2) + 0.00024178*dq4*cos(q2)*cos(q3)*sin(q5) - 0.0053163*dq4*cos(q4)*cos(q5)*sin(q2) + 0.00048356*dq5*cos(q2)*cos(q3)*sin(q5) + 0.00011114*dq5*cos(q2)*cos(q5)*sin(q3) - 0.00011114*dq5*cos(q3)*cos(q5)*sin(q2) - 0.0026581*dq5*cos(q4)*cos(q5)*sin(q2) - 0.000234*dq6*cos(q2)*cos(q3)*sin(q5) + 0.0010941*dq2*sin(q2)*sin(q3)*sin(q4) - 0.00011114*dq2*sin(q2)*sin(q3)*sin(q5) - 0.0010941*dq3*sin(q2)*sin(q3)*sin(q4) + 0.0013291*dq1*sin(q3)*sin(q4)*sin(q5) + 0.00011114*dq3*sin(q2)*sin(q3)*sin(q5) + 0.00024178*dq4*sin(q2)*sin(q3)*sin(q5) + 0.0026581*dq4*sin(q2)*sin(q4)*sin(q5) + 0.00048356*dq5*sin(q2)*sin(q3)*sin(q5) + 0.0053163*dq5*sin(q2)*sin(q4)*sin(q5) - 0.000234*dq6*sin(q2)*sin(q3)*sin(q5) + 0.0014978*dq1*cos(2.0*q2)*cos(2.0*q3)*sin(q5) + 0.0014978*dq1*sin(2.0*q2)*sin(2.0*q3)*sin(q5) - 0.002302*dq1*cos(2.0*q2)*cos(q3)*sin(q5) + 0.00065996*dq4*sin(2.0*q5)*cos(q2)*cos(q3) - 0.000060445*dq1*cos(2.0*q2)*cos(2.0*q3)*cos(2.0*q4)*sin(q5) - 0.00012089*dq1*cos(2.0*q2)*cos(2.0*q3)*sin(2.0*q4)*cos(q5) - 0.00076206*dq1*cos(2.0*q2)*cos(2.0*q5)*sin(2.0*q3)*cos(q4) + 0.00076206*dq1*cos(2.0*q3)*cos(2.0*q5)*sin(2.0*q2)*cos(q4) + 0.00038102*dq1*cos(2.0*q2)*sin(2.0*q3)*sin(2.0*q5)*sin(q4) - 0.00038102*dq1*cos(2.0*q3)*sin(2.0*q2)*sin(2.0*q5)*sin(q4) - 0.000060445*dq1*cos(2.0*q4)*sin(2.0*q2)*sin(2.0*q3)*sin(q5) - 0.00012089*dq1*sin(2.0*q2)*sin(2.0*q3)*sin(2.0*q4)*cos(q5) + 0.00041878*dq2*cos(q2)*cos(q3)*cos(q4)*sin(q5) + 1.5e-8*dq2*cos(q2)*cos(q3)*cos(q5)*sin(q4) + 0.00012839*dq2*cos(q2)*cos(q4)*cos(q5)*sin(q3) - 0.00012839*dq2*cos(q3)*cos(q4)*cos(q5)*sin(q2) - 0.00041878*dq3*cos(q2)*cos(q3)*cos(q4)*sin(q5) - 1.5e-8*dq3*cos(q2)*cos(q3)*cos(q5)*sin(q4) - 0.00012839*dq3*cos(q2)*cos(q4)*cos(q5)*sin(q3) + 0.00012839*dq3*cos(q3)*cos(q4)*cos(q5)*sin(q2) - 0.000064215*dq4*cos(q2)*cos(q3)*cos(q4)*sin(q5) - 0.00012839*dq4*cos(q2)*cos(q3)*cos(q5)*sin(q4) - 0.0033193*dq4*cos(q2)*cos(q4)*cos(q5)*sin(q3) + 0.0033193*dq4*cos(q3)*cos(q4)*cos(q5)*sin(q2) - 0.00012838*dq5*cos(q2)*cos(q3)*cos(q4)*sin(q5) - 0.00006422*dq5*cos(q2)*cos(q3)*cos(q5)*sin(q4) - 0.0020784*dq5*cos(q2)*cos(q4)*cos(q5)*sin(q3) + 0.0020784*dq5*cos(q3)*cos(q4)*cos(q5)*sin(q2) + 0.0002702*dq6*cos(q2)*cos(q4)*cos(q5)*sin(q3) - 0.0002702*dq6*cos(q3)*cos(q4)*cos(q5)*sin(q2) - 0.000064215*dq2*cos(q2)*sin(q3)*sin(q4)*sin(q5) + 0.000064215*dq2*cos(q3)*sin(q2)*sin(q4)*sin(q5) + 0.00041878*dq2*cos(q4)*sin(q2)*sin(q3)*sin(q5) + 1.5e-8*dq2*cos(q5)*sin(q2)*sin(q3)*sin(q4) + 0.000064215*dq3*cos(q2)*sin(q3)*sin(q4)*sin(q5) - 0.000064215*dq3*cos(q3)*sin(q2)*sin(q4)*sin(q5) - 0.00041878*dq3*cos(q4)*sin(q2)*sin(q3)*sin(q5) - 1.5e-8*dq3*cos(q5)*sin(q2)*sin(q3)*sin(q4) + 0.0016597*dq4*cos(q2)*sin(q3)*sin(q4)*sin(q5) - 0.0016597*dq4*cos(q3)*sin(q2)*sin(q4)*sin(q5) - 0.000064215*dq4*cos(q4)*sin(q2)*sin(q3)*sin(q5) - 0.00012839*dq4*cos(q5)*sin(q2)*sin(q3)*sin(q4) + 0.0033194*dq5*cos(q2)*sin(q3)*sin(q4)*sin(q5) - 0.0033194*dq5*cos(q3)*sin(q2)*sin(q4)*sin(q5) - 0.00012838*dq5*cos(q4)*sin(q2)*sin(q3)*sin(q5) - 0.00006422*dq5*cos(q5)*sin(q2)*sin(q3)*sin(q4) - 0.0001351*dq6*cos(q2)*sin(q3)*sin(q4)*sin(q5) + 0.0001351*dq6*cos(q3)*sin(q2)*sin(q4)*sin(q5) - 0.0016597*dq1*cos(2.0*q2)*sin(2.0*q3)*cos(q4)*cos(q5) + 0.0016597*dq1*cos(2.0*q3)*sin(2.0*q2)*cos(q4)*cos(q5) + 0.00043998*dq2*cos(2.0*q4)*cos(2.0*q5)*cos(q2)*sin(q3) - 0.00043998*dq2*cos(2.0*q4)*cos(2.0*q5)*cos(q3)*sin(q2) - 0.00043998*dq3*cos(2.0*q4)*cos(2.0*q5)*cos(q2)*sin(q3) + 0.00043998*dq3*cos(2.0*q4)*cos(2.0*q5)*cos(q3)*sin(q2) + 0.00062049*dq1*cos(2.0*q2)*sin(2.0*q3)*sin(q4)*sin(q5) - 0.00062049*dq1*cos(2.0*q3)*sin(2.0*q2)*sin(q4)*sin(q5) - 0.00054998*dq2*sin(2.0*q4)*sin(2.0*q5)*cos(q2)*sin(q3) + 0.00054998*dq2*sin(2.0*q4)*sin(2.0*q5)*cos(q3)*sin(q2) + 0.00054998*dq3*sin(2.0*q4)*sin(2.0*q5)*cos(q2)*sin(q3) - 0.00054998*dq3*sin(2.0*q4)*sin(2.0*q5)*cos(q3)*sin(q2) + 0.00027498*dq1*cos(2.0*q2)*cos(2.0*q3)*cos(2.0*q4)*sin(2.0*q5) + 0.00021998*dq1*cos(2.0*q2)*cos(2.0*q3)*cos(2.0*q5)*sin(2.0*q4) + 0.00027498*dq1*cos(2.0*q4)*sin(2.0*q2)*sin(2.0*q3)*sin(2.0*q5) + 0.00021998*dq1*cos(2.0*q5)*sin(2.0*q2)*sin(2.0*q3)*sin(2.0*q4) + 0.0026581*dq1*cos(2.0*q2)*cos(q4)*cos(q5)*sin(q3) - 0.0026581*dq1*sin(2.0*q2)*cos(q3)*cos(q4)*cos(q5) - 0.00024178*dq2*cos(2.0*q4)*cos(q2)*cos(q5)*sin(q3) + 0.00024178*dq2*cos(2.0*q4)*cos(q3)*cos(q5)*sin(q2) - 0.00076206*dq2*cos(2.0*q5)*cos(q2)*cos(q3)*sin(q4) - 0.00038102*dq2*sin(2.0*q5)*cos(q2)*cos(q3)*cos(q4) + 0.00024178*dq3*cos(2.0*q4)*cos(q2)*cos(q5)*sin(q3) - 0.00024178*dq3*cos(2.0*q4)*cos(q3)*cos(q5)*sin(q2) + 0.00076206*dq3*cos(2.0*q5)*cos(q2)*cos(q3)*sin(q4) + 0.00038102*dq3*sin(2.0*q5)*cos(q2)*cos(q3)*cos(q4) - 0.00076206*dq4*cos(2.0*q5)*cos(q2)*cos(q4)*sin(q3) + 0.00076206*dq4*cos(2.0*q5)*cos(q3)*cos(q4)*sin(q2) - 0.0013291*dq1*cos(2.0*q2)*sin(q3)*sin(q4)*sin(q5) + 0.0013291*dq1*sin(2.0*q2)*cos(q3)*sin(q4)*sin(q5) - 0.00076206*dq2*cos(2.0*q5)*sin(q2)*sin(q3)*sin(q4) + 0.00012089*dq2*sin(2.0*q4)*cos(q2)*sin(q3)*sin(q5) - 0.00012089*dq2*sin(2.0*q4)*cos(q3)*sin(q2)*sin(q5) - 0.00038102*dq2*sin(2.0*q5)*cos(q4)*sin(q2)*sin(q3) + 0.00076206*dq3*cos(2.0*q5)*sin(q2)*sin(q3)*sin(q4) - 0.00012089*dq3*sin(2.0*q4)*cos(q2)*sin(q3)*sin(q5) + 0.00012089*dq3*sin(2.0*q4)*cos(q3)*sin(q2)*sin(q5) + 0.00038102*dq3*sin(2.0*q5)*cos(q4)*sin(q2)*sin(q3) + 0.00038102*dq4*sin(2.0*q5)*cos(q2)*sin(q3)*sin(q4) - 0.00038102*dq4*sin(2.0*q5)*cos(q3)*sin(q2)*sin(q4);
 
C1_6 = 0.00010132*sin(q3 - 1.0*q2 + q4 + q5)*(dq3 - 1.0*dq2 + dq4 + dq5) - 0.00010132*sin(q2 - 1.0*q3 + q4 + q5)*(dq2 - 1.0*dq3 + dq4 + dq5) + 0.00006755*sin(q2 - 1.0*q3 + q4)*(dq2 - 1.0*dq3 + dq4) - 0.00006755*sin(q3 - 1.0*q2 + q4)*(dq3 - 1.0*dq2 + dq4) - 0.000117*sin(q2 - 1.0*q3 + q5)*(dq2 - 1.0*dq3 + dq5) - 0.000117*sin(q3 - 1.0*q2 + q5)*(dq3 - 1.0*dq2 + dq5) + 0.000033775*sin(q2 - 1.0*q3 + q4 - 1.0*q5)*(dq2 - 1.0*dq3 + dq4 - 1.0*dq5) - 0.000033775*sin(q2 - 1.0*q3 - 1.0*q4 + q5)*(dq2 - 1.0*dq3 - 1.0*dq4 + dq5) - 0.000078*sin(q2 - 1.0*q3)*(dq2 - 1.0*dq3);
 
C2_1 = 0.060795*dq1*sin(2.0*q2)*cos(q3) - 0.060795*dq1*cos(2.0*q2)*sin(q3) - 0.074028*dq1*sin(2.0*q2) - 2.0e-7*dq2*cos(q4)*sin(q2) - 0.0034398*dq4*cos(q2)*sin(q3) + 0.0034398*dq4*cos(q3)*sin(q2) - 0.017165*dq4*cos(q2)*sin(q4) - 0.0006317*dq5*cos(q2)*sin(q3) + 0.0006317*dq5*cos(q3)*sin(q2) - 0.000078*dq6*cos(q2)*sin(q3) + 0.000078*dq6*cos(q3)*sin(q2) + 0.018292*dq1*cos(2.0*q2)*sin(2.0*q3) - 0.018292*dq1*cos(2.0*q3)*sin(2.0*q2) - 0.017165*dq1*sin(2.0*q2)*sin(q3)*sin(q4) - 5.0e-8*dq2*sin(2.0*q4)*sin(q2)*sin(q3) + 5.0e-8*dq3*sin(2.0*q4)*sin(q2)*sin(q3) + 0.0010525*dq1*cos(2.0*q2)*cos(2.0*q4)*sin(2.0*q3) - 0.0010525*dq1*cos(2.0*q3)*cos(2.0*q4)*sin(2.0*q2) + 0.00049498*dq1*cos(2.0*q2)*cos(2.0*q5)*sin(2.0*q3) - 0.00049498*dq1*cos(2.0*q3)*cos(2.0*q5)*sin(2.0*q2) - 4.0e-8*dq2*cos(q2)*cos(q3)*sin(q4) - 2.0e-9*dq2*cos(q2)*cos(q5)*sin(q3) + 2.0e-9*dq2*cos(q3)*cos(q5)*sin(q2) + 4.0e-8*dq3*cos(q2)*cos(q3)*sin(q4) + 4.0e-8*dq2*cos(q4)*cos(q5)*sin(q2) + 2.0e-9*dq3*cos(q2)*cos(q5)*sin(q3) - 2.0e-9*dq3*cos(q3)*cos(q5)*sin(q2) + 0.010222*dq4*cos(q2)*cos(q3)*sin(q4) + 4.0e-8*dq4*cos(q2)*cos(q4)*sin(q3) - 4.0e-8*dq4*cos(q3)*cos(q4)*sin(q2) + 0.00024178*dq4*cos(q2)*cos(q5)*sin(q3) - 0.00024178*dq4*cos(q3)*cos(q5)*sin(q2) - 0.0010941*dq5*cos(q2)*cos(q3)*sin(q4) + 0.0053163*dq4*cos(q2)*cos(q4)*sin(q5) + 0.0026582*dq4*cos(q2)*cos(q5)*sin(q4) + 5.0e-9*dq5*cos(q2)*cos(q3)*sin(q5) + 0.00024178*dq5*cos(q2)*cos(q5)*sin(q3) - 0.00024178*dq5*cos(q3)*cos(q5)*sin(q2) - 0.0001351*dq6*cos(q2)*cos(q3)*sin(q4) + 0.0026582*dq5*cos(q2)*cos(q4)*sin(q5) + 0.0053163*dq5*cos(q2)*cos(q5)*sin(q4) - 0.000234*dq6*cos(q2)*cos(q5)*sin(q3) + 0.000234*dq6*cos(q3)*cos(q5)*sin(q2) - 4.0e-8*dq2*sin(q2)*sin(q3)*sin(q4) + 4.0e-8*dq3*sin(q2)*sin(q3)*sin(q4) - 6.0e-8*dq2*sin(q2)*sin(q4)*sin(q5) + 0.010222*dq4*sin(q2)*sin(q3)*sin(q4) - 0.0010941*dq5*sin(q2)*sin(q3)*sin(q4) + 5.0e-9*dq5*sin(q2)*sin(q3)*sin(q5) - 0.0001351*dq6*sin(q2)*sin(q3)*sin(q4) + 0.010222*dq1*cos(2.0*q2)*cos(2.0*q3)*sin(q4) + 0.0029956*dq1*cos(2.0*q2)*sin(2.0*q3)*cos(q5) - 0.0029956*dq1*cos(2.0*q3)*sin(2.0*q2)*cos(q5) + 0.010222*dq1*sin(2.0*q2)*sin(2.0*q3)*sin(q4) - 0.017165*dq1*cos(2.0*q2)*cos(q3)*sin(q4) - 0.004604*dq1*cos(2.0*q2)*cos(q5)*sin(q3) + 0.004604*dq1*sin(2.0*q2)*cos(q3)*cos(q5) - 5.0e-8*dq2*sin(2.0*q4)*cos(q2)*cos(q3) + 5.0e-8*dq3*sin(2.0*q4)*cos(q2)*cos(q3) + 0.0021051*dq4*cos(2.0*q4)*cos(q2)*sin(q3) - 0.0021051*dq4*cos(2.0*q4)*cos(q3)*sin(q2) + 0.00032998*dq4*cos(2.0*q5)*cos(q2)*sin(q3) - 0.00032998*dq4*cos(2.0*q5)*cos(q3)*sin(q2) - 0.00038102*dq1*cos(2.0*q2)*cos(2.0*q3)*cos(2.0*q5)*sin(q4) - 0.00076206*dq1*cos(2.0*q2)*cos(2.0*q3)*sin(2.0*q5)*cos(q4) - 0.00012089*dq1*cos(2.0*q2)*cos(2.0*q4)*sin(2.0*q3)*cos(q5) + 0.00012089*dq1*cos(2.0*q3)*cos(2.0*q4)*sin(2.0*q2)*cos(q5) + 0.00024178*dq1*cos(2.0*q2)*sin(2.0*q3)*sin(2.0*q4)*sin(q5) - 0.00024178*dq1*cos(2.0*q3)*sin(2.0*q2)*sin(2.0*q4)*sin(q5) - 0.00038102*dq1*cos(2.0*q5)*sin(2.0*q2)*sin(2.0*q3)*sin(q4) - 0.00076206*dq1*sin(2.0*q2)*sin(2.0*q3)*sin(2.0*q5)*cos(q4) + 3.0e-8*dq2*cos(q2)*cos(q3)*cos(q4)*sin(q5) + 2.35e-8*dq2*cos(q2)*cos(q3)*cos(q5)*sin(q4) + 1.5e-8*dq2*cos(q2)*cos(q4)*cos(q5)*sin(q3) - 1.5e-8*dq2*cos(q3)*cos(q4)*cos(q5)*sin(q2) - 3.0e-8*dq3*cos(q2)*cos(q3)*cos(q4)*sin(q5) - 2.35e-8*dq3*cos(q2)*cos(q3)*cos(q5)*sin(q4) - 1.5e-8*dq3*cos(q2)*cos(q4)*cos(q5)*sin(q3) + 1.5e-8*dq3*cos(q3)*cos(q4)*cos(q5)*sin(q2) - 0.0033194*dq4*cos(q2)*cos(q3)*cos(q4)*sin(q5) - 0.0012409*dq4*cos(q2)*cos(q3)*cos(q5)*sin(q4) - 2.35e-8*dq4*cos(q2)*cos(q4)*cos(q5)*sin(q3) + 2.35e-8*dq4*cos(q3)*cos(q4)*cos(q5)*sin(q2) - 0.0016597*dq5*cos(q2)*cos(q3)*cos(q4)*sin(q5) - 0.0033194*dq5*cos(q2)*cos(q3)*cos(q5)*sin(q4) - 2.5e-8*dq5*cos(q2)*cos(q4)*cos(q5)*sin(q3) + 2.5e-8*dq5*cos(q3)*cos(q4)*cos(q5)*sin(q2) + 0.0002702*dq6*cos(q2)*cos(q3)*cos(q4)*sin(q5) + 0.0001351*dq6*cos(q2)*cos(q3)*cos(q5)*sin(q4) - 3.5e-8*dq2*cos(q2)*sin(q3)*sin(q4)*sin(q5) + 3.5e-8*dq2*cos(q3)*sin(q2)*sin(q4)*sin(q5) + 3.0e-8*dq2*cos(q4)*sin(q2)*sin(q3)*sin(q5) + 2.35e-8*dq2*cos(q5)*sin(q2)*sin(q3)*sin(q4) + 3.5e-8*dq3*cos(q2)*sin(q3)*sin(q4)*sin(q5) - 3.5e-8*dq3*cos(q3)*sin(q2)*sin(q4)*sin(q5) - 3.0e-8*dq3*cos(q4)*sin(q2)*sin(q3)*sin(q5) - 2.35e-8*dq3*cos(q5)*sin(q2)*sin(q3)*sin(q4) + 3.0e-8*dq4*cos(q2)*sin(q3)*sin(q4)*sin(q5) - 3.0e-8*dq4*cos(q3)*sin(q2)*sin(q4)*sin(q5) - 0.0033194*dq4*cos(q4)*sin(q2)*sin(q3)*sin(q5) - 0.0012409*dq4*cos(q5)*sin(q2)*sin(q3)*sin(q4) + 2.85e-8*dq5*cos(q2)*sin(q3)*sin(q4)*sin(q5) - 2.85e-8*dq5*cos(q3)*sin(q2)*sin(q4)*sin(q5) - 0.0016597*dq5*cos(q4)*sin(q2)*sin(q3)*sin(q5) - 0.0033194*dq5*cos(q5)*sin(q2)*sin(q3)*sin(q4) + 0.0002702*dq6*cos(q4)*sin(q2)*sin(q3)*sin(q5) + 0.0001351*dq6*cos(q5)*sin(q2)*sin(q3)*sin(q4) - 0.0033194*dq1*cos(2.0*q2)*cos(2.0*q3)*cos(q4)*sin(q5) - 0.001241*dq1*cos(2.0*q2)*cos(2.0*q3)*cos(q5)*sin(q4) + 2.0e-9*dq2*cos(2.0*q4)*sin(2.0*q5)*cos(q2)*cos(q3) + 3.0e-9*dq2*cos(2.0*q5)*sin(2.0*q4)*cos(q2)*cos(q3) - 2.0e-9*dq3*cos(2.0*q4)*sin(2.0*q5)*cos(q2)*cos(q3) - 3.0e-9*dq3*cos(2.0*q5)*sin(2.0*q4)*cos(q2)*cos(q3) + 0.00054997*dq4*cos(2.0*q4)*cos(2.0*q5)*cos(q2)*sin(q3) - 0.00054997*dq4*cos(2.0*q4)*cos(2.0*q5)*cos(q3)*sin(q2) + 0.00043998*dq5*cos(2.0*q4)*cos(2.0*q5)*cos(q2)*sin(q3) - 0.00043998*dq5*cos(2.0*q4)*cos(2.0*q5)*cos(q3)*sin(q2) - 0.0033194*dq1*sin(2.0*q2)*sin(2.0*q3)*cos(q4)*sin(q5) - 0.001241*dq1*sin(2.0*q2)*sin(2.0*q3)*cos(q5)*sin(q4) + 2.0e-9*dq2*cos(2.0*q4)*sin(2.0*q5)*sin(q2)*sin(q3) + 3.0e-9*dq2*cos(2.0*q5)*sin(2.0*q4)*sin(q2)*sin(q3) - 2.0e-9*dq3*cos(2.0*q4)*sin(2.0*q5)*sin(q2)*sin(q3) - 3.0e-9*dq3*cos(2.0*q5)*sin(2.0*q4)*sin(q2)*sin(q3) - 0.00043998*dq4*sin(2.0*q4)*sin(2.0*q5)*cos(q2)*sin(q3) + 0.00043998*dq4*sin(2.0*q4)*sin(2.0*q5)*cos(q3)*sin(q2) - 0.00054997*dq5*sin(2.0*q4)*sin(2.0*q5)*cos(q2)*sin(q3) + 0.00054997*dq5*sin(2.0*q4)*sin(2.0*q5)*cos(q3)*sin(q2) + 0.00027498*dq1*cos(2.0*q2)*cos(2.0*q4)*cos(2.0*q5)*sin(2.0*q3) - 0.00027498*dq1*cos(2.0*q3)*cos(2.0*q4)*cos(2.0*q5)*sin(2.0*q2) - 0.00021998*dq1*cos(2.0*q2)*sin(2.0*q3)*sin(2.0*q4)*sin(2.0*q5) + 0.00021998*dq1*cos(2.0*q3)*sin(2.0*q2)*sin(2.0*q4)*sin(2.0*q5) + 0.0053163*dq1*cos(2.0*q2)*cos(q3)*cos(q4)*sin(q5) + 0.0026581*dq1*cos(2.0*q2)*cos(q3)*cos(q5)*sin(q4) - 5.0e-9*dq2*cos(2.0*q4)*cos(q2)*cos(q3)*sin(q5) + 3.0e-9*dq2*cos(2.0*q5)*cos(q2)*cos(q4)*sin(q3) - 3.0e-9*dq2*cos(2.0*q5)*cos(q3)*cos(q4)*sin(q2) - 5.0e-9*dq2*sin(2.0*q4)*cos(q2)*cos(q3)*cos(q5) + 5.0e-9*dq3*cos(2.0*q4)*cos(q2)*cos(q3)*sin(q5) - 3.0e-9*dq3*cos(2.0*q5)*cos(q2)*cos(q4)*sin(q3) + 3.0e-9*dq3*cos(2.0*q5)*cos(q3)*cos(q4)*sin(q2) + 5.0e-9*dq3*sin(2.0*q4)*cos(q2)*cos(q3)*cos(q5) - 0.00024178*dq4*cos(2.0*q4)*cos(q2)*cos(q5)*sin(q3) + 0.00024178*dq4*cos(2.0*q4)*cos(q3)*cos(q5)*sin(q2) - 0.00038103*dq4*cos(2.0*q5)*cos(q2)*cos(q3)*sin(q4) - 0.00076206*dq4*sin(2.0*q5)*cos(q2)*cos(q3)*cos(q4) - 0.00024178*dq5*cos(2.0*q4)*cos(q2)*cos(q5)*sin(q3) + 0.00024178*dq5*cos(2.0*q4)*cos(q3)*cos(q5)*sin(q2) - 0.00076206*dq5*cos(2.0*q5)*cos(q2)*cos(q3)*sin(q4) - 0.00038103*dq5*sin(2.0*q5)*cos(q2)*cos(q3)*cos(q4) + 0.0053163*dq1*sin(2.0*q2)*cos(q4)*sin(q3)*sin(q5) + 0.0026581*dq1*sin(2.0*q2)*cos(q5)*sin(q3)*sin(q4) - 5.0e-9*dq2*cos(2.0*q4)*sin(q2)*sin(q3)*sin(q5) - 5.0e-9*dq2*sin(2.0*q4)*cos(q5)*sin(q2)*sin(q3) - 2.0e-9*dq2*sin(2.0*q5)*cos(q2)*sin(q3)*sin(q4) + 2.0e-9*dq2*sin(2.0*q5)*cos(q3)*sin(q2)*sin(q4) + 5.0e-9*dq3*cos(2.0*q4)*sin(q2)*sin(q3)*sin(q5) + 5.0e-9*dq3*sin(2.0*q4)*cos(q5)*sin(q2)*sin(q3) + 2.0e-9*dq3*sin(2.0*q5)*cos(q2)*sin(q3)*sin(q4) - 2.0e-9*dq3*sin(2.0*q5)*cos(q3)*sin(q2)*sin(q4) - 0.00038103*dq4*cos(2.0*q5)*sin(q2)*sin(q3)*sin(q4) + 0.00048356*dq4*sin(2.0*q4)*cos(q2)*sin(q3)*sin(q5) - 0.00048356*dq4*sin(2.0*q4)*cos(q3)*sin(q2)*sin(q5) - 0.00076206*dq4*sin(2.0*q5)*cos(q4)*sin(q2)*sin(q3) - 0.00076206*dq5*cos(2.0*q5)*sin(q2)*sin(q3)*sin(q4) + 0.00012089*dq5*sin(2.0*q4)*cos(q2)*sin(q3)*sin(q5) - 0.00012089*dq5*sin(2.0*q4)*cos(q3)*sin(q2)*sin(q5) - 0.00038103*dq5*sin(2.0*q5)*cos(q4)*sin(q2)*sin(q3);
 
C2_2 = 0.0021051*dq4*sin(2.0*q4) - 0.00032998*dq5*sin(2.0*q5) + 0.060795*dq3*sin(q3) - 0.0027538*dq5*sin(q5) - 0.00048356*dq4*cos(2.0*q4)*sin(q5) - 0.00024178*dq4*sin(2.0*q4)*cos(q5) - 0.00012089*dq5*cos(2.0*q4)*sin(q5) - 0.00024178*dq5*sin(2.0*q4)*cos(q5) + 0.017164*dq3*cos(q3)*sin(q4) + 0.0046041*dq3*cos(q5)*sin(q3) + 0.017164*dq4*cos(q4)*sin(q3) + 0.0046041*dq5*cos(q3)*sin(q5) + 0.00043998*dq4*cos(2.0*q4)*sin(2.0*q5) + 0.00054997*dq4*cos(2.0*q5)*sin(2.0*q4) + 0.00054997*dq5*cos(2.0*q4)*sin(2.0*q5) + 0.00043998*dq5*cos(2.0*q5)*sin(2.0*q4) - 0.0053165*dq3*cos(q3)*cos(q4)*sin(q5) - 0.0026582*dq3*cos(q3)*cos(q5)*sin(q4) - 0.0026582*dq4*cos(q4)*cos(q5)*sin(q3) - 0.0053165*dq5*cos(q4)*cos(q5)*sin(q3) + 0.0053165*dq4*sin(q3)*sin(q4)*sin(q5) + 0.0026582*dq5*sin(q3)*sin(q4)*sin(q5);
 
C2_3 = 0.00043998*dq4*sin(2.0*q5) - 0.0015551*dq4*sin(2.0*q4) + 0.00043998*dq5*sin(2.0*q4) + 0.00087995*dq5*sin(2.0*q5) + 0.060795*dq2*sin(q3) - 0.060795*dq3*sin(q3) - 0.00048356*dq4*sin(q5) + 0.0026329*dq5*sin(q5) + 0.017164*dq2*cos(q3)*sin(q4) + 0.0046041*dq2*cos(q5)*sin(q3) - 0.017165*dq3*cos(q3)*sin(q4) - 0.0046041*dq3*cos(q5)*sin(q3) - 0.017165*dq4*cos(q4)*sin(q3) - 0.0046041*dq5*cos(q3)*sin(q5) + 0.00096712*dq4*cos(q4)^2*sin(q5) + 0.00024178*dq5*cos(q4)^2*sin(q5) - 0.0053165*dq2*cos(q3)*cos(q4)*sin(q5) - 0.0026582*dq2*cos(q3)*cos(q5)*sin(q4) + 0.0053164*dq3*cos(q3)*cos(q4)*sin(q5) + 0.0026582*dq3*cos(q3)*cos(q5)*sin(q4) + 0.0026582*dq4*cos(q4)*cos(q5)*sin(q3) + 0.00048356*dq4*cos(q4)*cos(q5)*sin(q4) + 0.0053164*dq5*cos(q4)*cos(q5)*sin(q3) + 0.00048356*dq5*cos(q4)*cos(q5)*sin(q4) - 0.0053164*dq4*sin(q3)*sin(q4)*sin(q5) - 0.0026582*dq5*sin(q3)*sin(q4)*sin(q5) - 0.0021999*dq4*cos(q4)*cos(q5)^2*sin(q4) - 0.0017599*dq4*cos(q4)^2*cos(q5)*sin(q5) - 0.0017599*dq5*cos(q4)*cos(q5)^2*sin(q4) - 0.0021999*dq5*cos(q4)^2*cos(q5)*sin(q5);
 
C2_4 = 0.0021051*dq2*sin(2.0*q4) - 0.0021051*dq3*sin(2.0*q4) + 0.010222*dq4*sin(q4) - 0.0010941*dq5*sin(q4) - 0.0001351*dq6*sin(q4) - 0.00048356*dq2*cos(2.0*q4)*sin(q5) - 0.00024178*dq2*sin(2.0*q4)*cos(q5) + 0.00048356*dq3*cos(2.0*q4)*sin(q5) + 0.00024178*dq3*sin(2.0*q4)*cos(q5) - 0.00038103*dq4*cos(2.0*q5)*sin(q4) - 0.00076206*dq4*sin(2.0*q5)*cos(q4) - 0.00076206*dq5*cos(2.0*q5)*sin(q4) - 0.00038103*dq5*sin(2.0*q5)*cos(q4) - 0.0034398*dq1*cos(q2)*sin(q3) + 0.0034398*dq1*cos(q3)*sin(q2) - 0.017165*dq1*cos(q2)*sin(q4) + 0.017164*dq2*cos(q4)*sin(q3) - 0.017165*dq3*cos(q4)*sin(q3) - 0.017165*dq4*cos(q3)*sin(q4) - 0.0033194*dq4*cos(q4)*sin(q5) - 0.0012409*dq4*cos(q5)*sin(q4) - 0.0016597*dq5*cos(q4)*sin(q5) - 0.0033194*dq5*cos(q5)*sin(q4) + 0.0002702*dq6*cos(q4)*sin(q5) + 0.0001351*dq6*cos(q5)*sin(q4) + 0.00043998*dq2*cos(2.0*q4)*sin(2.0*q5) + 0.00054997*dq2*cos(2.0*q5)*sin(2.0*q4) - 0.00043998*dq3*cos(2.0*q4)*sin(2.0*q5) - 0.00054997*dq3*cos(2.0*q5)*sin(2.0*q4) + 0.010222*dq1*cos(q2)*cos(q3)*sin(q4) + 0.00024178*dq1*cos(q2)*cos(q5)*sin(q3) - 0.00024178*dq1*cos(q3)*cos(q5)*sin(q2) + 0.0053164*dq1*cos(q2)*cos(q4)*sin(q5) + 0.0026582*dq1*cos(q2)*cos(q5)*sin(q4) - 0.0026582*dq2*cos(q4)*cos(q5)*sin(q3) + 0.0026582*dq3*cos(q4)*cos(q5)*sin(q3) + 0.0053164*dq4*cos(q3)*cos(q4)*sin(q5) + 0.0026582*dq4*cos(q3)*cos(q5)*sin(q4) + 0.0026582*dq5*cos(q3)*cos(q4)*sin(q5) + 0.0053164*dq5*cos(q3)*cos(q5)*sin(q4) + 0.010222*dq1*sin(q2)*sin(q3)*sin(q4) + 0.0053165*dq2*sin(q3)*sin(q4)*sin(q5) - 0.0053164*dq3*sin(q3)*sin(q4)*sin(q5) + 0.0021051*dq1*cos(2.0*q4)*cos(q2)*sin(q3) - 0.0021051*dq1*cos(2.0*q4)*cos(q3)*sin(q2) + 0.00032998*dq1*cos(2.0*q5)*cos(q2)*sin(q3) - 0.00032998*dq1*cos(2.0*q5)*cos(q3)*sin(q2) - 0.0033194*dq1*cos(q2)*cos(q3)*cos(q4)*sin(q5) - 0.0012409*dq1*cos(q2)*cos(q3)*cos(q5)*sin(q4) - 0.0033194*dq1*cos(q4)*sin(q2)*sin(q3)*sin(q5) - 0.0012409*dq1*cos(q5)*sin(q2)*sin(q3)*sin(q4) + 0.00054997*dq1*cos(2.0*q4)*cos(2.0*q5)*cos(q2)*sin(q3) - 0.00054997*dq1*cos(2.0*q4)*cos(2.0*q5)*cos(q3)*sin(q2) - 0.00043998*dq1*sin(2.0*q4)*sin(2.0*q5)*cos(q2)*sin(q3) + 0.00043998*dq1*sin(2.0*q4)*sin(2.0*q5)*cos(q3)*sin(q2) - 0.00024178*dq1*cos(2.0*q4)*cos(q2)*cos(q5)*sin(q3) + 0.00024178*dq1*cos(2.0*q4)*cos(q3)*cos(q5)*sin(q2) - 0.00038103*dq1*cos(2.0*q5)*cos(q2)*cos(q3)*sin(q4) - 0.00076206*dq1*sin(2.0*q5)*cos(q2)*cos(q3)*cos(q4) - 0.00038103*dq1*cos(2.0*q5)*sin(q2)*sin(q3)*sin(q4) + 0.00048356*dq1*sin(2.0*q4)*cos(q2)*sin(q3)*sin(q5) - 0.00048356*dq1*sin(2.0*q4)*cos(q3)*sin(q2)*sin(q5) - 0.00076206*dq1*sin(2.0*q5)*cos(q4)*sin(q2)*sin(q3);
 
C2_5 = 0.00032998*dq3*sin(2.0*q5) - 0.00032998*dq2*sin(2.0*q5) - 0.0027538*dq2*sin(q5) + 0.0027538*dq3*sin(q5) - 0.0010941*dq4*sin(q4) + 0.5*dq6*(0.0002702*cos(q4)*sin(q5) + 0.0005404*cos(q5)*sin(q4)) - 0.00012089*dq2*cos(2.0*q4)*sin(q5) - 0.00024178*dq2*sin(2.0*q4)*cos(q5) + 0.00012089*dq3*cos(2.0*q4)*sin(q5) + 0.00024178*dq3*sin(2.0*q4)*cos(q5) - 0.00076206*dq4*cos(2.0*q5)*sin(q4) - 0.00038103*dq4*sin(2.0*q5)*cos(q4) - 0.0006317*dq1*cos(q2)*sin(q3) + 0.0006317*dq1*cos(q3)*sin(q2) + 0.0046041*dq2*cos(q3)*sin(q5) - 0.0046041*dq3*cos(q3)*sin(q5) - 0.0016597*dq4*cos(q4)*sin(q5) - 0.0033194*dq4*cos(q5)*sin(q4) - 0.0046041*dq5*cos(q5)*sin(q3) - 0.0033194*dq5*cos(q4)*sin(q5) - 0.0020785*dq5*cos(q5)*sin(q4) + 0.00054997*dq2*cos(2.0*q4)*sin(2.0*q5) + 0.00043998*dq2*cos(2.0*q5)*sin(2.0*q4) - 0.00054997*dq3*cos(2.0*q4)*sin(2.0*q5) - 0.00043998*dq3*cos(2.0*q5)*sin(2.0*q4) - 0.0010941*dq1*cos(q2)*cos(q3)*sin(q4) + 0.00024178*dq1*cos(q2)*cos(q5)*sin(q3) - 0.00024178*dq1*cos(q3)*cos(q5)*sin(q2) + 0.0026582*dq1*cos(q2)*cos(q4)*sin(q5) + 0.0053164*dq1*cos(q2)*cos(q5)*sin(q4) - 0.0053165*dq2*cos(q4)*cos(q5)*sin(q3) + 0.0053164*dq3*cos(q4)*cos(q5)*sin(q3) + 0.0026582*dq4*cos(q3)*cos(q4)*sin(q5) + 0.0053164*dq4*cos(q3)*cos(q5)*sin(q4) + 0.0053164*dq5*cos(q3)*cos(q4)*sin(q5) + 0.0026582*dq5*cos(q3)*cos(q5)*sin(q4) - 0.0010941*dq1*sin(q2)*sin(q3)*sin(q4) + 0.0026582*dq2*sin(q3)*sin(q4)*sin(q5) - 0.0026582*dq3*sin(q3)*sin(q4)*sin(q5) - 0.0016597*dq1*cos(q2)*cos(q3)*cos(q4)*sin(q5) - 0.0033194*dq1*cos(q2)*cos(q3)*cos(q5)*sin(q4) - 0.0016597*dq1*cos(q4)*sin(q2)*sin(q3)*sin(q5) - 0.0033194*dq1*cos(q5)*sin(q2)*sin(q3)*sin(q4) + 0.00043998*dq1*cos(2.0*q4)*cos(2.0*q5)*cos(q2)*sin(q3) - 0.00043998*dq1*cos(2.0*q4)*cos(2.0*q5)*cos(q3)*sin(q2) - 0.00054997*dq1*sin(2.0*q4)*sin(2.0*q5)*cos(q2)*sin(q3) + 0.00054997*dq1*sin(2.0*q4)*sin(2.0*q5)*cos(q3)*sin(q2) - 0.00024178*dq1*cos(2.0*q4)*cos(q2)*cos(q5)*sin(q3) + 0.00024178*dq1*cos(2.0*q4)*cos(q3)*cos(q5)*sin(q2) - 0.00076206*dq1*cos(2.0*q5)*cos(q2)*cos(q3)*sin(q4) - 0.00038103*dq1*sin(2.0*q5)*cos(q2)*cos(q3)*cos(q4) - 0.00076206*dq1*cos(2.0*q5)*sin(q2)*sin(q3)*sin(q4) + 0.00012089*dq1*sin(2.0*q4)*cos(q2)*sin(q3)*sin(q5) - 0.00012089*dq1*sin(2.0*q4)*cos(q3)*sin(q2)*sin(q5) - 0.00038103*dq1*sin(2.0*q5)*cos(q4)*sin(q2)*sin(q3);
 
C2_6 = 0.000078*dq1*sin(q2 - 1.0*q3) - 0.0001351*dq4*sin(q4) + 0.0002702*dq4*cos(q4)*sin(q5) + 0.0001351*dq4*cos(q5)*sin(q4) + 0.0001351*dq5*cos(q4)*sin(q5) + 0.0002702*dq5*cos(q5)*sin(q4) - 0.0001351*dq1*cos(q2 - 1.0*q3)*sin(q4) + 0.000234*dq1*sin(q2 - 1.0*q3)*cos(q5) + 0.0002702*dq1*cos(q2 - 1.0*q3)*cos(q4)*sin(q5) + 0.0001351*dq1*cos(q2 - 1.0*q3)*cos(q5)*sin(q4);
 
C3_1 = 0.0042912*dq1*sin(q3 - 1.0*q4) - 0.001151*dq1*sin(q3 - 1.0*q5) - 0.0034398*dq4*sin(q2 - 1.0*q3) - 0.0006317*dq5*sin(q2 - 1.0*q3) - 0.000078*dq6*sin(q2 - 1.0*q3) + 0.0042912*dq1*sin(2.0*q2 - 1.0*q3 + q4) - 0.005111*dq1*sin(2.0*q3 - 2.0*q2 + q4) - 0.001151*dq1*sin(2.0*q2 - 1.0*q3 + q5) - 0.005111*dq1*sin(2.0*q2 - 2.0*q3 + q4) + 2.5e-8*dq2*sin(q2 - 1.0*q3 + 2.0*q4) + 2.5e-8*dq2*sin(q3 - 1.0*q2 + 2.0*q4) - 0.0014978*dq1*sin(2.0*q3 - 2.0*q2 + q5) + 0.0014978*dq1*sin(2.0*q2 - 2.0*q3 + q5) - 2.5e-8*dq3*sin(q2 - 1.0*q3 + 2.0*q4) - 2.5e-8*dq3*sin(q3 - 1.0*q2 + 2.0*q4) + 0.0010526*dq4*sin(q2 - 1.0*q3 + 2.0*q4) - 0.0010526*dq4*sin(q3 - 1.0*q2 + 2.0*q4) + 0.00016499*dq4*sin(q2 - 1.0*q3 + 2.0*q5) - 0.00016499*dq4*sin(q3 - 1.0*q2 + 2.0*q5) + 0.00033227*dq1*sin(2.0*q2 - 1.0*q3 + q4 - 1.0*q5) - 0.00033227*dq1*sin(2.0*q2 - 1.0*q3 - 1.0*q4 + q5) - 0.00051961*dq1*sin(2.0*q2 - 2.0*q3 + q4 - 1.0*q5) + 0.00051961*dq1*sin(2.0*q2 - 2.0*q3 - 1.0*q4 + q5) + 2.5e-10*dq2*sin(q2 - 1.0*q3 - 1.0*q4 + 2.0*q5) + 0.00028577*dq1*sin(2.0*q3 - 2.0*q2 + q4 + 2.0*q5) + 0.000090668*dq1*sin(2.0*q3 - 2.0*q2 + 2.0*q4 + q5) - 0.000095258*dq1*sin(2.0*q2 - 2.0*q3 + q4 - 2.0*q5) + 0.00028577*dq1*sin(2.0*q2 - 2.0*q3 + q4 + 2.0*q5) + 0.000030223*dq1*sin(2.0*q2 - 2.0*q3 - 2.0*q4 + q5) - 0.000090668*dq1*sin(2.0*q2 - 2.0*q3 + 2.0*q4 + q5) + 2.5e-10*dq2*sin(q2 - 1.0*q3 - 2.0*q4 + 2.0*q5) - 2.5e-10*dq2*sin(q2 - 1.0*q3 + 2.0*q4 - 2.0*q5) - 1.25e-9*dq2*sin(q2 - 1.0*q3 + 2.0*q4 + 2.0*q5) - 1.25e-9*dq2*sin(q3 - 1.0*q2 + 2.0*q4 + 2.0*q5) - 2.5e-10*dq3*sin(q2 - 1.0*q3 - 1.0*q4 + 2.0*q5) - 2.5e-10*dq3*sin(q2 - 1.0*q3 - 2.0*q4 + 2.0*q5) + 2.5e-10*dq3*sin(q2 - 1.0*q3 + 2.0*q4 - 2.0*q5) + 1.25e-9*dq3*sin(q2 - 1.0*q3 + 2.0*q4 + 2.0*q5) + 1.25e-9*dq3*sin(q3 - 1.0*q2 + 2.0*q4 + 2.0*q5) + 0.000095258*dq4*sin(q2 - 1.0*q3 - 1.0*q4 + 2.0*q5) + 0.000060445*dq4*sin(q2 - 1.0*q3 + 2.0*q4 - 1.0*q5) + 0.000027498*dq4*sin(q2 - 1.0*q3 - 2.0*q4 + 2.0*q5) + 0.000027498*dq4*sin(q2 - 1.0*q3 + 2.0*q4 - 2.0*q5) + 0.00024749*dq4*sin(q2 - 1.0*q3 + 2.0*q4 + 2.0*q5) - 0.00024749*dq4*sin(q3 - 1.0*q2 + 2.0*q4 + 2.0*q5) - 0.000095258*dq5*sin(q2 - 1.0*q3 - 1.0*q4 + 2.0*q5) - 0.000030222*dq5*sin(q2 - 1.0*q3 + 2.0*q4 - 1.0*q5) - 0.000027498*dq5*sin(q2 - 1.0*q3 - 2.0*q4 + 2.0*q5) - 0.000027498*dq5*sin(q2 - 1.0*q3 + 2.0*q4 - 2.0*q5) + 0.00024749*dq5*sin(q2 - 1.0*q3 + 2.0*q4 + 2.0*q5) - 0.00024749*dq5*sin(q3 - 1.0*q2 + 2.0*q4 + 2.0*q5) - 0.0042912*dq1*sin(q3 + q4) - 0.001151*dq1*sin(q3 + q5) + 0.0042912*dq1*sin(q3 - 2.0*q2 + q4) + 2.0e-8*dq2*sin(q2 - 1.0*q3 + q4) + 2.0e-8*dq2*sin(q3 - 1.0*q2 + q4) + 0.001151*dq1*sin(q3 - 2.0*q2 + q5) - 1.0e-9*dq2*sin(q2 - 1.0*q3 + q5) + 1.0e-9*dq2*sin(q3 - 1.0*q2 + q5) - 2.0e-8*dq3*sin(q2 - 1.0*q3 + q4) - 2.0e-8*dq3*sin(q3 - 1.0*q2 + q4) - 0.00033227*dq1*sin(q3 + q4 - 1.0*q5) + 0.00033227*dq1*sin(q3 - 1.0*q4 + q5) + 0.0009968*dq1*sin(q4 - 1.0*q3 + q5) + 1.0e-9*dq3*sin(q2 - 1.0*q3 + q5) - 1.0e-9*dq3*sin(q3 - 1.0*q2 + q5) - 0.005111*dq4*sin(q2 - 1.0*q3 + q4) - 0.005111*dq4*sin(q3 - 1.0*q2 + q4) + 0.00012089*dq4*sin(q2 - 1.0*q3 + q5) - 0.00012089*dq4*sin(q3 - 1.0*q2 + q5) + 0.00054705*dq5*sin(q2 - 1.0*q3 + q4) + 0.00054705*dq5*sin(q3 - 1.0*q2 + q4) + 0.00012089*dq5*sin(q2 - 1.0*q3 + q5) - 0.00012089*dq5*sin(q3 - 1.0*q2 + q5) + 0.00006755*dq6*sin(q2 - 1.0*q3 + q4) + 0.00006755*dq6*sin(q3 - 1.0*q2 + q4) - 0.000117*dq6*sin(q2 - 1.0*q3 + q5) + 0.000117*dq6*sin(q3 - 1.0*q2 + q5) - 0.0009968*dq1*sin(2.0*q2 - 1.0*q3 + q4 + q5) - 3.375e-9*dq2*sin(q2 - 1.0*q3 + q4 - 1.0*q5) - 6.625e-9*dq2*sin(q2 - 1.0*q3 - 1.0*q4 + q5) + 0.0011401*dq1*sin(2.0*q3 - 2.0*q2 + q4 + q5) + 0.0011401*dq1*sin(2.0*q2 - 2.0*q3 + q4 + q5) + 2.5e-10*dq2*sin(q2 - 1.0*q3 + q4 - 2.0*q5) + 1.25e-9*dq2*sin(q2 - 1.0*q3 + q4 + 2.0*q5) + 2.5e-9*dq2*sin(q2 - 1.0*q3 + 2.0*q4 + q5) - 1.25e-9*dq2*sin(q3 - 1.0*q2 + q4 + 2.0*q5) + 2.5e-9*dq2*sin(q3 - 1.0*q2 + 2.0*q4 + q5) + 3.375e-9*dq3*sin(q2 - 1.0*q3 + q4 - 1.0*q5) + 6.625e-9*dq3*sin(q2 - 1.0*q3 - 1.0*q4 + q5) - 2.5e-10*dq3*sin(q2 - 1.0*q3 + q4 - 2.0*q5) - 1.25e-9*dq3*sin(q2 - 1.0*q3 + q4 + 2.0*q5) - 2.5e-9*dq3*sin(q2 - 1.0*q3 + 2.0*q4 + q5) + 1.25e-9*dq3*sin(q3 - 1.0*q2 + q4 + 2.0*q5) - 2.5e-9*dq3*sin(q3 - 1.0*q2 + 2.0*q4 + q5) - 0.00051962*dq4*sin(q2 - 1.0*q3 + q4 - 1.0*q5) + 0.00051962*dq4*sin(q2 - 1.0*q3 - 1.0*q4 + q5) - 0.000095258*dq4*sin(q2 - 1.0*q3 + q4 - 2.0*q5) + 0.00028577*dq4*sin(q2 - 1.0*q3 + q4 + 2.0*q5) + 0.000060445*dq4*sin(q2 - 1.0*q3 - 2.0*q4 + q5) - 0.00018134*dq4*sin(q2 - 1.0*q3 + 2.0*q4 + q5) + 0.00028577*dq4*sin(q3 - 1.0*q2 + q4 + 2.0*q5) + 0.00018134*dq4*sin(q3 - 1.0*q2 + 2.0*q4 + q5) + 0.00041493*dq5*sin(q2 - 1.0*q3 + q4 - 1.0*q5) - 0.00041493*dq5*sin(q2 - 1.0*q3 - 1.0*q4 + q5) + 0.000095258*dq5*sin(q2 - 1.0*q3 + q4 - 2.0*q5) + 0.00028577*dq5*sin(q2 - 1.0*q3 + q4 + 2.0*q5) - 0.000030222*dq5*sin(q2 - 1.0*q3 - 2.0*q4 + q5) - 0.000090668*dq5*sin(q2 - 1.0*q3 + 2.0*q4 + q5) + 0.00028577*dq5*sin(q3 - 1.0*q2 + q4 + 2.0*q5) + 0.000090668*dq5*sin(q3 - 1.0*q2 + 2.0*q4 + q5) + 0.000033775*dq6*sin(q2 - 1.0*q3 + q4 - 1.0*q5) - 0.000033775*dq6*sin(q2 - 1.0*q3 - 1.0*q4 + q5) - 0.030397*dq1*sin(q3) - 0.030397*dq1*sin(2.0*q2 - 1.0*q3) + 0.018292*dq1*sin(2.0*q2 - 2.0*q3) - 0.00052627*dq1*sin(2.0*q3 - 2.0*q2 + 2.0*q4) + 0.00052627*dq1*sin(2.0*q2 - 2.0*q3 + 2.0*q4) - 0.00024749*dq1*sin(2.0*q3 - 2.0*q2 + 2.0*q5) + 0.00024749*dq1*sin(2.0*q2 - 2.0*q3 + 2.0*q5) + 0.000095258*dq1*sin(2.0*q2 - 2.0*q3 - 1.0*q4 + 2.0*q5) + 0.000030223*dq1*sin(2.0*q2 - 2.0*q3 + 2.0*q4 - 1.0*q5) - 0.00012374*dq1*sin(2.0*q3 - 2.0*q2 + 2.0*q4 + 2.0*q5) + 0.000013749*dq1*sin(2.0*q2 - 2.0*q3 - 2.0*q4 + 2.0*q5) + 0.000013749*dq1*sin(2.0*q2 - 2.0*q3 + 2.0*q4 - 2.0*q5) + 0.00012374*dq1*sin(2.0*q2 - 2.0*q3 + 2.0*q4 + 2.0*q5) + 0.0009968*dq1*sin(q3 + q4 + q5) - 0.0009968*dq1*sin(q3 - 2.0*q2 + q4 + q5) - 8.75e-10*dq2*sin(q2 - 1.0*q3 + q4 + q5) - 2.5875e-8*dq2*sin(q3 - 1.0*q2 + q4 + q5) + 8.75e-10*dq3*sin(q2 - 1.0*q3 + q4 + q5) + 2.5875e-8*dq3*sin(q3 - 1.0*q2 + q4 + q5) + 0.00114*dq4*sin(q2 - 1.0*q3 + q4 + q5) + 0.0011401*dq4*sin(q3 - 1.0*q2 + q4 + q5) + 0.0012447*dq5*sin(q2 - 1.0*q3 + q4 + q5) + 0.0012448*dq5*sin(q3 - 1.0*q2 + q4 + q5) - 0.00010132*dq6*sin(q2 - 1.0*q3 + q4 + q5) - 0.00010132*dq6*sin(q3 - 1.0*q2 + q4 + q5);
 
C3_2 = 0.00043998*dq4*sin(2.0*q5) - 0.0015551*dq4*sin(2.0*q4) + 0.00043998*dq5*sin(2.0*q4) + 0.00087995*dq5*sin(2.0*q5) - 0.060795*dq2*sin(q3) - 0.00048356*dq4*sin(q5) + 0.0026329*dq5*sin(q5) - 0.017164*dq2*cos(q3)*sin(q4) - 0.0046041*dq2*cos(q5)*sin(q3) + 0.00096712*dq4*cos(q4)^2*sin(q5) + 0.00024178*dq5*cos(q4)^2*sin(q5) + 0.0053165*dq2*cos(q3)*cos(q4)*sin(q5) + 0.0026582*dq2*cos(q3)*cos(q5)*sin(q4) + 0.00048356*dq4*cos(q4)*cos(q5)*sin(q4) + 0.00048356*dq5*cos(q4)*cos(q5)*sin(q4) - 0.0021999*dq4*cos(q4)*cos(q5)^2*sin(q4) - 0.0017599*dq4*cos(q4)^2*cos(q5)*sin(q5) - 0.0017599*dq5*cos(q4)*cos(q5)^2*sin(q4) - 0.0021999*dq5*cos(q4)^2*cos(q5)*sin(q5);
 
C3_3 = 0.0021051*dq4*sin(2.0*q4) - 0.00032998*dq5*sin(2.0*q5) - 0.0027538*dq5*sin(q5) - 0.00048356*dq4*cos(2.0*q4)*sin(q5) - 0.00024178*dq4*sin(2.0*q4)*cos(q5) - 0.00012089*dq5*cos(2.0*q4)*sin(q5) - 0.00024178*dq5*sin(2.0*q4)*cos(q5) + 0.00043998*dq4*cos(2.0*q4)*sin(2.0*q5) + 0.00054997*dq4*cos(2.0*q5)*sin(2.0*q4) + 0.00054997*dq5*cos(2.0*q4)*sin(2.0*q5) + 0.00043998*dq5*cos(2.0*q5)*sin(2.0*q4);
 
C3_4 = 0.0021051*dq3*sin(2.0*q4) - 0.0021051*dq2*sin(2.0*q4) - 0.010222*dq4*sin(q4) + 0.0010941*dq5*sin(q4) + 0.0001351*dq6*sin(q4) + 0.00048356*dq2*cos(2.0*q4)*sin(q5) + 0.00024178*dq2*sin(2.0*q4)*cos(q5) - 0.00048356*dq3*cos(2.0*q4)*sin(q5) - 0.00024178*dq3*sin(2.0*q4)*cos(q5) + 0.00038103*dq4*cos(2.0*q5)*sin(q4) + 0.00076206*dq4*sin(2.0*q5)*cos(q4) + 0.00076206*dq5*cos(2.0*q5)*sin(q4) + 0.00038103*dq5*sin(2.0*q5)*cos(q4) + 0.0034398*dq1*cos(q2)*sin(q3) - 0.0034398*dq1*cos(q3)*sin(q2) + 0.0033194*dq4*cos(q4)*sin(q5) + 0.0012409*dq4*cos(q5)*sin(q4) + 0.0016597*dq5*cos(q4)*sin(q5) + 0.0033194*dq5*cos(q5)*sin(q4) - 0.0002702*dq6*cos(q4)*sin(q5) - 0.0001351*dq6*cos(q5)*sin(q4) - 0.00043998*dq2*cos(2.0*q4)*sin(2.0*q5) - 0.00054997*dq2*cos(2.0*q5)*sin(2.0*q4) + 0.00043998*dq3*cos(2.0*q4)*sin(2.0*q5) + 0.00054997*dq3*cos(2.0*q5)*sin(2.0*q4) - 0.010222*dq1*cos(q2)*cos(q3)*sin(q4) - 0.00024178*dq1*cos(q2)*cos(q5)*sin(q3) + 0.00024178*dq1*cos(q3)*cos(q5)*sin(q2) - 0.010222*dq1*sin(q2)*sin(q3)*sin(q4) - 0.0021051*dq1*cos(2.0*q4)*cos(q2)*sin(q3) + 0.0021051*dq1*cos(2.0*q4)*cos(q3)*sin(q2) - 0.00032998*dq1*cos(2.0*q5)*cos(q2)*sin(q3) + 0.00032998*dq1*cos(2.0*q5)*cos(q3)*sin(q2) + 0.0033194*dq1*cos(q2)*cos(q3)*cos(q4)*sin(q5) + 0.0012409*dq1*cos(q2)*cos(q3)*cos(q5)*sin(q4) + 0.0033194*dq1*cos(q4)*sin(q2)*sin(q3)*sin(q5) + 0.0012409*dq1*cos(q5)*sin(q2)*sin(q3)*sin(q4) - 0.00054997*dq1*cos(2.0*q4)*cos(2.0*q5)*cos(q2)*sin(q3) + 0.00054997*dq1*cos(2.0*q4)*cos(2.0*q5)*cos(q3)*sin(q2) + 0.00043998*dq1*sin(2.0*q4)*sin(2.0*q5)*cos(q2)*sin(q3) - 0.00043998*dq1*sin(2.0*q4)*sin(2.0*q5)*cos(q3)*sin(q2) + 0.00024178*dq1*cos(2.0*q4)*cos(q2)*cos(q5)*sin(q3) - 0.00024178*dq1*cos(2.0*q4)*cos(q3)*cos(q5)*sin(q2) + 0.00038103*dq1*cos(2.0*q5)*cos(q2)*cos(q3)*sin(q4) + 0.00076206*dq1*sin(2.0*q5)*cos(q2)*cos(q3)*cos(q4) + 0.00038103*dq1*cos(2.0*q5)*sin(q2)*sin(q3)*sin(q4) - 0.00048356*dq1*sin(2.0*q4)*cos(q2)*sin(q3)*sin(q5) + 0.00048356*dq1*sin(2.0*q4)*cos(q3)*sin(q2)*sin(q5) + 0.00076206*dq1*sin(2.0*q5)*cos(q4)*sin(q2)*sin(q3);
 
C3_5 = 0.00032998*dq2*sin(2.0*q5) - 0.00032998*dq3*sin(2.0*q5) + 0.0027538*dq2*sin(q5) - 0.0027538*dq3*sin(q5) + 0.0010941*dq4*sin(q4) + 0.00012089*dq2*cos(2.0*q4)*sin(q5) + 0.00024178*dq2*sin(2.0*q4)*cos(q5) - 0.00012089*dq3*cos(2.0*q4)*sin(q5) - 0.00024178*dq3*sin(2.0*q4)*cos(q5) + 0.00076206*dq4*cos(2.0*q5)*sin(q4) + 0.00038103*dq4*sin(2.0*q5)*cos(q4) + 0.0006317*dq1*cos(q2)*sin(q3) - 0.0006317*dq1*cos(q3)*sin(q2) + 0.0016597*dq4*cos(q4)*sin(q5) + 0.0033194*dq4*cos(q5)*sin(q4) + 0.0033194*dq5*cos(q4)*sin(q5) + 0.0020785*dq5*cos(q5)*sin(q4) - 0.0001351*dq6*cos(q4)*sin(q5) - 0.0002702*dq6*cos(q5)*sin(q4) - 0.00054997*dq2*cos(2.0*q4)*sin(2.0*q5) - 0.00043998*dq2*cos(2.0*q5)*sin(2.0*q4) + 0.00054997*dq3*cos(2.0*q4)*sin(2.0*q5) + 0.00043998*dq3*cos(2.0*q5)*sin(2.0*q4) + 0.0010941*dq1*cos(q2)*cos(q3)*sin(q4) - 0.00024178*dq1*cos(q2)*cos(q5)*sin(q3) + 0.00024178*dq1*cos(q3)*cos(q5)*sin(q2) + 0.0010941*dq1*sin(q2)*sin(q3)*sin(q4) + 0.0016597*dq1*cos(q2)*cos(q3)*cos(q4)*sin(q5) + 0.0033194*dq1*cos(q2)*cos(q3)*cos(q5)*sin(q4) + 0.0016597*dq1*cos(q4)*sin(q2)*sin(q3)*sin(q5) + 0.0033194*dq1*cos(q5)*sin(q2)*sin(q3)*sin(q4) - 0.00043998*dq1*cos(2.0*q4)*cos(2.0*q5)*cos(q2)*sin(q3) + 0.00043998*dq1*cos(2.0*q4)*cos(2.0*q5)*cos(q3)*sin(q2) + 0.00054997*dq1*sin(2.0*q4)*sin(2.0*q5)*cos(q2)*sin(q3) - 0.00054997*dq1*sin(2.0*q4)*sin(2.0*q5)*cos(q3)*sin(q2) + 0.00024178*dq1*cos(2.0*q4)*cos(q2)*cos(q5)*sin(q3) - 0.00024178*dq1*cos(2.0*q4)*cos(q3)*cos(q5)*sin(q2) + 0.00076206*dq1*cos(2.0*q5)*cos(q2)*cos(q3)*sin(q4) + 0.00038103*dq1*sin(2.0*q5)*cos(q2)*cos(q3)*cos(q4) + 0.00076206*dq1*cos(2.0*q5)*sin(q2)*sin(q3)*sin(q4) - 0.00012089*dq1*sin(2.0*q4)*cos(q2)*sin(q3)*sin(q5) + 0.00012089*dq1*sin(2.0*q4)*cos(q3)*sin(q2)*sin(q5) + 0.00038103*dq1*sin(2.0*q5)*cos(q4)*sin(q2)*sin(q3);
 
C3_6 = 0.0001351*dq4*sin(q4) - 0.000078*dq1*sin(q2 - 1.0*q3) - 0.0002702*dq4*cos(q4)*sin(q5) - 0.0001351*dq4*cos(q5)*sin(q4) - 0.0001351*dq5*cos(q4)*sin(q5) - 0.0002702*dq5*cos(q5)*sin(q4) + 0.0001351*dq1*cos(q2 - 1.0*q3)*sin(q4) - 0.000234*dq1*sin(q2 - 1.0*q3)*cos(q5) - 0.0002702*dq1*cos(q2 - 1.0*q3)*cos(q4)*sin(q5) - 0.0001351*dq1*cos(q2 - 1.0*q3)*cos(q5)*sin(q4);
 
C4_1 = 0.0010525*dq1*sin(2.0*q4) - 0.00041432*dq1*sin(q4) - 0.00024178*dq1*cos(2.0*q4)*sin(q5) - 0.00012089*dq1*sin(2.0*q4)*cos(q5) + 0.0034398*dq2*cos(q2)*sin(q3) - 0.0034398*dq2*cos(q3)*sin(q2) - 0.0085823*dq1*cos(q4)*sin(q3) + 0.017165*dq2*cos(q2)*sin(q4) - 0.0034398*dq3*cos(q2)*sin(q3) + 0.0034398*dq3*cos(q3)*sin(q2) + 0.00012833*dq1*cos(q4)*sin(q5) + 0.000064164*dq1*cos(q5)*sin(q4) + 2.0e-7*dq4*cos(q4)*sin(q2) + 0.00021999*dq1*cos(2.0*q4)*sin(2.0*q5) + 0.00027499*dq1*cos(2.0*q5)*sin(2.0*q4) + 0.00065996*dq5*sin(2.0*q5)*sin(q2)*sin(q3) - 0.0010525*dq1*cos(2.0*q2)*cos(2.0*q3)*sin(2.0*q4) - 0.0010525*dq1*sin(2.0*q2)*sin(2.0*q3)*sin(2.0*q4) - 0.010222*dq2*cos(q2)*cos(q3)*sin(q4) + 4.0e-8*dq2*cos(q2)*cos(q4)*sin(q3) - 4.0e-8*dq2*cos(q3)*cos(q4)*sin(q2) - 0.00024178*dq2*cos(q2)*cos(q5)*sin(q3) + 0.00024178*dq2*cos(q3)*cos(q5)*sin(q2) + 0.010222*dq3*cos(q2)*cos(q3)*sin(q4) - 4.0e-8*dq3*cos(q2)*cos(q4)*sin(q3) + 4.0e-8*dq3*cos(q3)*cos(q4)*sin(q2) + 0.0013291*dq1*cos(q4)*cos(q5)*sin(q3) - 0.0053163*dq2*cos(q2)*cos(q4)*sin(q5) - 0.0026582*dq2*cos(q2)*cos(q5)*sin(q4) + 0.00024178*dq3*cos(q2)*cos(q5)*sin(q3) - 0.00024178*dq3*cos(q3)*cos(q5)*sin(q2) - 4.0e-8*dq4*cos(q2)*cos(q3)*sin(q4) + 0.0010941*dq5*cos(q2)*cos(q4)*sin(q3) - 0.0010941*dq5*cos(q3)*cos(q4)*sin(q2) - 4.0e-8*dq4*cos(q4)*cos(q5)*sin(q2) + 0.00024178*dq5*cos(q2)*cos(q3)*sin(q5) + 0.0001351*dq6*cos(q2)*cos(q4)*sin(q3) - 0.0001351*dq6*cos(q3)*cos(q4)*sin(q2) - 6.0e-8*dq5*cos(q4)*cos(q5)*sin(q2) - 0.010222*dq2*sin(q2)*sin(q3)*sin(q4) + 0.010222*dq3*sin(q2)*sin(q3)*sin(q4) - 0.0026581*dq1*sin(q3)*sin(q4)*sin(q5) - 4.0e-8*dq4*sin(q2)*sin(q3)*sin(q4) + 6.0e-8*dq4*sin(q2)*sin(q4)*sin(q5) + 0.00024178*dq5*sin(q2)*sin(q3)*sin(q5) + 4.0e-8*dq5*sin(q2)*sin(q4)*sin(q5) - 0.005111*dq1*cos(2.0*q2)*sin(2.0*q3)*cos(q4) + 0.005111*dq1*cos(2.0*q3)*sin(2.0*q2)*cos(q4) + 0.0085823*dq1*cos(2.0*q2)*cos(q4)*sin(q3) - 0.0085823*dq1*sin(2.0*q2)*cos(q3)*cos(q4) - 0.002105*dq2*cos(2.0*q4)*cos(q2)*sin(q3) + 0.002105*dq2*cos(2.0*q4)*cos(q3)*sin(q2) - 0.00032998*dq2*cos(2.0*q5)*cos(q2)*sin(q3) + 0.00032998*dq2*cos(2.0*q5)*cos(q3)*sin(q2) + 0.002105*dq3*cos(2.0*q4)*cos(q2)*sin(q3) - 0.002105*dq3*cos(2.0*q4)*cos(q3)*sin(q2) + 0.00032998*dq3*cos(2.0*q5)*cos(q2)*sin(q3) - 0.00032998*dq3*cos(2.0*q5)*cos(q3)*sin(q2) + 0.00065996*dq5*sin(2.0*q5)*cos(q2)*cos(q3) + 0.00024178*dq1*cos(2.0*q2)*cos(2.0*q3)*cos(2.0*q4)*sin(q5) + 0.00012089*dq1*cos(2.0*q2)*cos(2.0*q3)*sin(2.0*q4)*cos(q5) + 0.00019051*dq1*cos(2.0*q2)*cos(2.0*q5)*sin(2.0*q3)*cos(q4) - 0.00019051*dq1*cos(2.0*q3)*cos(2.0*q5)*sin(2.0*q2)*cos(q4) - 0.00038103*dq1*cos(2.0*q2)*sin(2.0*q3)*sin(2.0*q5)*sin(q4) + 0.00038103*dq1*cos(2.0*q3)*sin(2.0*q2)*sin(2.0*q5)*sin(q4) + 0.00024178*dq1*cos(2.0*q4)*sin(2.0*q2)*sin(2.0*q3)*sin(q5) + 0.00012089*dq1*sin(2.0*q2)*sin(2.0*q3)*sin(2.0*q4)*cos(q5) + 0.0033194*dq2*cos(q2)*cos(q3)*cos(q4)*sin(q5) + 0.0012409*dq2*cos(q2)*cos(q3)*cos(q5)*sin(q4) - 2.35e-8*dq2*cos(q2)*cos(q4)*cos(q5)*sin(q3) + 2.35e-8*dq2*cos(q3)*cos(q4)*cos(q5)*sin(q2) - 0.0033194*dq3*cos(q2)*cos(q3)*cos(q4)*sin(q5) - 0.0012409*dq3*cos(q2)*cos(q3)*cos(q5)*sin(q4) + 2.35e-8*dq3*cos(q2)*cos(q4)*cos(q5)*sin(q3) - 2.35e-8*dq3*cos(q3)*cos(q4)*cos(q5)*sin(q2) + 3.0e-8*dq4*cos(q2)*cos(q3)*cos(q4)*sin(q5) + 2.35e-8*dq4*cos(q2)*cos(q3)*cos(q5)*sin(q4) - 1.5e-8*dq4*cos(q2)*cos(q4)*cos(q5)*sin(q3) + 1.5e-8*dq4*cos(q3)*cos(q4)*cos(q5)*sin(q2) + 2.85e-8*dq5*cos(q2)*cos(q3)*cos(q4)*sin(q5) + 2.5e-8*dq5*cos(q2)*cos(q3)*cos(q5)*sin(q4) - 2.0e-8*dq5*cos(q2)*cos(q4)*cos(q5)*sin(q3) + 2.0e-8*dq5*cos(q3)*cos(q4)*cos(q5)*sin(q2) - 0.0001351*dq6*cos(q2)*cos(q4)*cos(q5)*sin(q3) + 0.0001351*dq6*cos(q3)*cos(q4)*cos(q5)*sin(q2) + 3.0e-8*dq2*cos(q2)*sin(q3)*sin(q4)*sin(q5) - 3.0e-8*dq2*cos(q3)*sin(q2)*sin(q4)*sin(q5) + 0.0033194*dq2*cos(q4)*sin(q2)*sin(q3)*sin(q5) + 0.0012409*dq2*cos(q5)*sin(q2)*sin(q3)*sin(q4) - 3.0e-8*dq3*cos(q2)*sin(q3)*sin(q4)*sin(q5) + 3.0e-8*dq3*cos(q3)*sin(q2)*sin(q4)*sin(q5) - 0.0033194*dq3*cos(q4)*sin(q2)*sin(q3)*sin(q5) - 0.0012409*dq3*cos(q5)*sin(q2)*sin(q3)*sin(q4) + 3.5e-8*dq4*cos(q2)*sin(q3)*sin(q4)*sin(q5) - 3.5e-8*dq4*cos(q3)*sin(q2)*sin(q4)*sin(q5) + 3.0e-8*dq4*cos(q4)*sin(q2)*sin(q3)*sin(q5) + 2.35e-8*dq4*cos(q5)*sin(q2)*sin(q3)*sin(q4) - 0.00041877*dq5*cos(q2)*sin(q3)*sin(q4)*sin(q5) + 0.00041877*dq5*cos(q3)*sin(q2)*sin(q4)*sin(q5) + 2.85e-8*dq5*cos(q4)*sin(q2)*sin(q3)*sin(q5) + 2.5e-8*dq5*cos(q5)*sin(q2)*sin(q3)*sin(q4) + 0.0002702*dq6*cos(q2)*sin(q3)*sin(q4)*sin(q5) - 0.0002702*dq6*cos(q3)*sin(q2)*sin(q4)*sin(q5) + 0.00062049*dq1*cos(2.0*q2)*sin(2.0*q3)*cos(q4)*cos(q5) - 0.00062049*dq1*cos(2.0*q3)*sin(2.0*q2)*cos(q4)*cos(q5) - 0.00054998*dq2*cos(2.0*q4)*cos(2.0*q5)*cos(q2)*sin(q3) + 0.00054998*dq2*cos(2.0*q4)*cos(2.0*q5)*cos(q3)*sin(q2) + 0.00054998*dq3*cos(2.0*q4)*cos(2.0*q5)*cos(q2)*sin(q3) - 0.00054998*dq3*cos(2.0*q4)*cos(2.0*q5)*cos(q3)*sin(q2) - 0.0016597*dq1*cos(2.0*q2)*sin(2.0*q3)*sin(q4)*sin(q5) + 0.0016597*dq1*cos(2.0*q3)*sin(2.0*q2)*sin(q4)*sin(q5) + 0.00043998*dq2*sin(2.0*q4)*sin(2.0*q5)*cos(q2)*sin(q3) - 0.00043998*dq2*sin(2.0*q4)*sin(2.0*q5)*cos(q3)*sin(q2) - 0.00043998*dq3*sin(2.0*q4)*sin(2.0*q5)*cos(q2)*sin(q3) + 0.00043998*dq3*sin(2.0*q4)*sin(2.0*q5)*cos(q3)*sin(q2) - 0.00021998*dq1*cos(2.0*q2)*cos(2.0*q3)*cos(2.0*q4)*sin(2.0*q5) - 0.00027498*dq1*cos(2.0*q2)*cos(2.0*q3)*cos(2.0*q5)*sin(2.0*q4) - 0.00021998*dq1*cos(2.0*q4)*sin(2.0*q2)*sin(2.0*q3)*sin(2.0*q5) - 0.00027498*dq1*cos(2.0*q5)*sin(2.0*q2)*sin(2.0*q3)*sin(2.0*q4) - 0.0013291*dq1*cos(2.0*q2)*cos(q4)*cos(q5)*sin(q3) + 0.0013291*dq1*sin(2.0*q2)*cos(q3)*cos(q4)*cos(q5) + 0.00024179*dq2*cos(2.0*q4)*cos(q2)*cos(q5)*sin(q3) - 0.00024179*dq2*cos(2.0*q4)*cos(q3)*cos(q5)*sin(q2) + 0.00038103*dq2*cos(2.0*q5)*cos(q2)*cos(q3)*sin(q4) + 0.00076206*dq2*sin(2.0*q5)*cos(q2)*cos(q3)*cos(q4) - 0.00024179*dq3*cos(2.0*q4)*cos(q2)*cos(q5)*sin(q3) + 0.00024179*dq3*cos(2.0*q4)*cos(q3)*cos(q5)*sin(q2) - 0.00038103*dq3*cos(2.0*q5)*cos(q2)*cos(q3)*sin(q4) - 0.00076206*dq3*sin(2.0*q5)*cos(q2)*cos(q3)*cos(q4) - 3.0e-9*dq4*cos(2.0*q5)*cos(q2)*cos(q4)*sin(q3) + 3.0e-9*dq4*cos(2.0*q5)*cos(q3)*cos(q4)*sin(q2) - 0.00076206*dq5*cos(2.0*q5)*cos(q2)*cos(q4)*sin(q3) + 0.00076206*dq5*cos(2.0*q5)*cos(q3)*cos(q4)*sin(q2) + 0.0026581*dq1*cos(2.0*q2)*sin(q3)*sin(q4)*sin(q5) - 0.0026581*dq1*sin(2.0*q2)*cos(q3)*sin(q4)*sin(q5) + 0.00038103*dq2*cos(2.0*q5)*sin(q2)*sin(q3)*sin(q4) - 0.00048357*dq2*sin(2.0*q4)*cos(q2)*sin(q3)*sin(q5) + 0.00048357*dq2*sin(2.0*q4)*cos(q3)*sin(q2)*sin(q5) + 0.00076206*dq2*sin(2.0*q5)*cos(q4)*sin(q2)*sin(q3) - 0.00038103*dq3*cos(2.0*q5)*sin(q2)*sin(q3)*sin(q4) + 0.00048357*dq3*sin(2.0*q4)*cos(q2)*sin(q3)*sin(q5) - 0.00048357*dq3*sin(2.0*q4)*cos(q3)*sin(q2)*sin(q5) - 0.00076206*dq3*sin(2.0*q5)*cos(q4)*sin(q2)*sin(q3) + 2.0e-9*dq4*sin(2.0*q5)*cos(q2)*sin(q3)*sin(q4) - 2.0e-9*dq4*sin(2.0*q5)*cos(q3)*sin(q2)*sin(q4) + 0.00038103*dq5*sin(2.0*q5)*cos(q2)*sin(q3)*sin(q4) - 0.00038103*dq5*sin(2.0*q5)*cos(q3)*sin(q2)*sin(q4);
 
C4_2 = 0.0021051*dq3*sin(2.0*q4) - 0.0021051*dq2*sin(2.0*q4) + 0.0010941*dq5*sin(q4) + 0.0001351*dq6*sin(q4) + 0.00048356*dq2*cos(2.0*q4)*sin(q5) + 0.00024178*dq2*sin(2.0*q4)*cos(q5) - 0.00048356*dq3*cos(2.0*q4)*sin(q5) - 0.00024178*dq3*sin(2.0*q4)*cos(q5) - 0.00076206*dq5*cos(2.0*q5)*sin(q4) - 0.00038103*dq5*sin(2.0*q5)*cos(q4) + 0.0034398*dq1*cos(q2)*sin(q3) - 0.0034398*dq1*cos(q3)*sin(q2) + 0.017165*dq1*cos(q2)*sin(q4) - 0.017164*dq2*cos(q4)*sin(q3) + 0.0004188*dq5*cos(q4)*sin(q5) - 0.0002702*dq6*cos(q4)*sin(q5) - 0.0001351*dq6*cos(q5)*sin(q4) - 0.00043998*dq2*cos(2.0*q4)*sin(2.0*q5) - 0.00054997*dq2*cos(2.0*q5)*sin(2.0*q4) + 0.00043998*dq3*cos(2.0*q4)*sin(2.0*q5) + 0.00054997*dq3*cos(2.0*q5)*sin(2.0*q4) - 0.010222*dq1*cos(q2)*cos(q3)*sin(q4) - 0.00024178*dq1*cos(q2)*cos(q5)*sin(q3) + 0.00024178*dq1*cos(q3)*cos(q5)*sin(q2) - 0.0053164*dq1*cos(q2)*cos(q4)*sin(q5) - 0.0026582*dq1*cos(q2)*cos(q5)*sin(q4) + 0.0026582*dq2*cos(q4)*cos(q5)*sin(q3) - 0.010222*dq1*sin(q2)*sin(q3)*sin(q4) - 0.0053165*dq2*sin(q3)*sin(q4)*sin(q5) - 0.0021051*dq1*cos(2.0*q4)*cos(q2)*sin(q3) + 0.0021051*dq1*cos(2.0*q4)*cos(q3)*sin(q2) - 0.00032998*dq1*cos(2.0*q5)*cos(q2)*sin(q3) + 0.00032998*dq1*cos(2.0*q5)*cos(q3)*sin(q2) + 0.0033194*dq1*cos(q2)*cos(q3)*cos(q4)*sin(q5) + 0.0012409*dq1*cos(q2)*cos(q3)*cos(q5)*sin(q4) + 0.0033194*dq1*cos(q4)*sin(q2)*sin(q3)*sin(q5) + 0.0012409*dq1*cos(q5)*sin(q2)*sin(q3)*sin(q4) - 0.00054997*dq1*cos(2.0*q4)*cos(2.0*q5)*cos(q2)*sin(q3) + 0.00054997*dq1*cos(2.0*q4)*cos(2.0*q5)*cos(q3)*sin(q2) + 0.00043998*dq1*sin(2.0*q4)*sin(2.0*q5)*cos(q2)*sin(q3) - 0.00043998*dq1*sin(2.0*q4)*sin(2.0*q5)*cos(q3)*sin(q2) + 0.00024178*dq1*cos(2.0*q4)*cos(q2)*cos(q5)*sin(q3) - 0.00024178*dq1*cos(2.0*q4)*cos(q3)*cos(q5)*sin(q2) + 0.00038103*dq1*cos(2.0*q5)*cos(q2)*cos(q3)*sin(q4) + 0.00076206*dq1*sin(2.0*q5)*cos(q2)*cos(q3)*cos(q4) + 0.00038103*dq1*cos(2.0*q5)*sin(q2)*sin(q3)*sin(q4) - 0.00048356*dq1*sin(2.0*q4)*cos(q2)*sin(q3)*sin(q5) + 0.00048356*dq1*sin(2.0*q4)*cos(q3)*sin(q2)*sin(q5) + 0.00076206*dq1*sin(2.0*q5)*cos(q4)*sin(q2)*sin(q3);
 
C4_3 = 0.0021051*dq2*sin(2.0*q4) - 0.0021051*dq3*sin(2.0*q4) - 0.0010941*dq5*sin(q4) - 0.0001351*dq6*sin(q4) - 0.00048356*dq2*cos(2.0*q4)*sin(q5) - 0.00024178*dq2*sin(2.0*q4)*cos(q5) + 0.00048356*dq3*cos(2.0*q4)*sin(q5) + 0.00024178*dq3*sin(2.0*q4)*cos(q5) + 0.00076206*dq5*cos(2.0*q5)*sin(q4) + 0.00038103*dq5*sin(2.0*q5)*cos(q4) - 0.0034398*dq1*cos(q2)*sin(q3) + 0.0034398*dq1*cos(q3)*sin(q2) - 0.0004188*dq5*cos(q4)*sin(q5) + 0.0002702*dq6*cos(q4)*sin(q5) + 0.0001351*dq6*cos(q5)*sin(q4) + 0.00043998*dq2*cos(2.0*q4)*sin(2.0*q5) + 0.00054997*dq2*cos(2.0*q5)*sin(2.0*q4) - 0.00043998*dq3*cos(2.0*q4)*sin(2.0*q5) - 0.00054997*dq3*cos(2.0*q5)*sin(2.0*q4) + 0.010222*dq1*cos(q2)*cos(q3)*sin(q4) + 0.00024178*dq1*cos(q2)*cos(q5)*sin(q3) - 0.00024178*dq1*cos(q3)*cos(q5)*sin(q2) + 0.010222*dq1*sin(q2)*sin(q3)*sin(q4) + 0.0021051*dq1*cos(2.0*q4)*cos(q2)*sin(q3) - 0.0021051*dq1*cos(2.0*q4)*cos(q3)*sin(q2) + 0.00032998*dq1*cos(2.0*q5)*cos(q2)*sin(q3) - 0.00032998*dq1*cos(2.0*q5)*cos(q3)*sin(q2) - 0.0033194*dq1*cos(q2)*cos(q3)*cos(q4)*sin(q5) - 0.0012409*dq1*cos(q2)*cos(q3)*cos(q5)*sin(q4) - 0.0033194*dq1*cos(q4)*sin(q2)*sin(q3)*sin(q5) - 0.0012409*dq1*cos(q5)*sin(q2)*sin(q3)*sin(q4) + 0.00054997*dq1*cos(2.0*q4)*cos(2.0*q5)*cos(q2)*sin(q3) - 0.00054997*dq1*cos(2.0*q4)*cos(2.0*q5)*cos(q3)*sin(q2) - 0.00043998*dq1*sin(2.0*q4)*sin(2.0*q5)*cos(q2)*sin(q3) + 0.00043998*dq1*sin(2.0*q4)*sin(2.0*q5)*cos(q3)*sin(q2) - 0.00024178*dq1*cos(2.0*q4)*cos(q2)*cos(q5)*sin(q3) + 0.00024178*dq1*cos(2.0*q4)*cos(q3)*cos(q5)*sin(q2) - 0.00038103*dq1*cos(2.0*q5)*cos(q2)*cos(q3)*sin(q4) - 0.00076206*dq1*sin(2.0*q5)*cos(q2)*cos(q3)*cos(q4) - 0.00038103*dq1*cos(2.0*q5)*sin(q2)*sin(q3)*sin(q4) + 0.00048356*dq1*sin(2.0*q4)*cos(q2)*sin(q3)*sin(q5) - 0.00048356*dq1*sin(2.0*q4)*cos(q3)*sin(q2)*sin(q5) - 0.00076206*dq1*sin(2.0*q5)*cos(q4)*sin(q2)*sin(q3);
 
C4_4 = 2.7105e-20*dq5*(2.4348e+16*sin(2.0*q5) + 8.9201e+15*sin(q5));
 
C4_5 = 0.5*dq4*(0.0013199*sin(2.0*q5) + 0.00048356*sin(q5)) + 0.0018562*dq2*sin(q4) - 0.0018562*dq3*sin(q4) + 0.00048356*dq5*sin(q5) - 0.000234*dq6*sin(q5) + 0.0004188*dq2*cos(q4)*sin(q5) - 0.0004188*dq3*cos(q4)*sin(q5) - 0.0015241*dq2*cos(q5)^2*sin(q4) + 0.0015241*dq3*cos(q5)^2*sin(q4) + 0.0018562*dq1*cos(q2)*cos(q4)*sin(q3) - 0.0018562*dq1*cos(q3)*cos(q4)*sin(q2) + 0.00024178*dq1*cos(q2)*cos(q3)*sin(q5) - 0.00076206*dq2*cos(q4)*cos(q5)*sin(q5) + 0.00076206*dq3*cos(q4)*cos(q5)*sin(q5) + 0.00024178*dq1*sin(q2)*sin(q3)*sin(q5) + 0.0013199*dq1*cos(q2)*cos(q3)*cos(q5)*sin(q5) - 0.0004188*dq1*cos(q2)*sin(q3)*sin(q4)*sin(q5) + 0.0004188*dq1*cos(q3)*sin(q2)*sin(q4)*sin(q5) + 0.0013199*dq1*cos(q5)*sin(q2)*sin(q3)*sin(q5) - 0.0015241*dq1*cos(q2)*cos(q4)*cos(q5)^2*sin(q3) + 0.0015241*dq1*cos(q3)*cos(q4)*cos(q5)^2*sin(q2) + 0.00076206*dq1*cos(q2)*cos(q5)*sin(q3)*sin(q4)*sin(q5) - 0.00076206*dq1*cos(q3)*cos(q5)*sin(q2)*sin(q4)*sin(q5);
 
C4_6 = 0.0001351*dq3*(2.0*cos(q4)*sin(q5) - 1.0*sin(q4) + cos(q5)*sin(q4)) - 0.0001351*dq2*(2.0*cos(q4)*sin(q5) - 1.0*sin(q4) + cos(q5)*sin(q4)) - 0.000234*dq5*sin(q5) - 0.0001351*dq1*sin(q2 - 1.0*q3)*(cos(q4) - 1.0*cos(q4)*cos(q5) + 2.0*sin(q4)*sin(q5));
 
C5_1 = 0.001256*dq1*sin(q5) - 0.00016499*dq1*sin(2.0*q5) - 0.000060447*dq1*cos(2.0*q4)*sin(q5) - 0.00012089*dq1*sin(2.0*q4)*cos(q5) + 0.0006317*dq2*cos(q2)*sin(q3) - 0.0006317*dq2*cos(q3)*sin(q2) - 0.0006317*dq3*cos(q2)*sin(q3) + 0.0006317*dq3*cos(q3)*sin(q2) - 0.002302*dq1*cos(q3)*sin(q5) + 0.000064164*dq1*cos(q4)*sin(q5) + 0.00012833*dq1*cos(q5)*sin(q4) + 0.00027499*dq1*cos(2.0*q4)*sin(2.0*q5) + 0.00021999*dq1*cos(2.0*q5)*sin(2.0*q4) + 0.002302*dq1*sin(2.0*q2)*sin(q3)*sin(q5) - 0.00065996*dq4*sin(2.0*q5)*sin(q2)*sin(q3) - 0.00049498*dq1*cos(2.0*q2)*cos(2.0*q3)*sin(2.0*q5) - 0.00049498*dq1*sin(2.0*q2)*sin(2.0*q3)*sin(2.0*q5) + 0.0010941*dq2*cos(q2)*cos(q3)*sin(q4) + 2.0e-9*dq2*cos(q2)*cos(q3)*sin(q5) - 0.00024178*dq2*cos(q2)*cos(q5)*sin(q3) + 0.00024178*dq2*cos(q3)*cos(q5)*sin(q2) - 0.0010941*dq3*cos(q2)*cos(q3)*sin(q4) + 0.0026581*dq1*cos(q4)*cos(q5)*sin(q3) - 0.0026582*dq2*cos(q2)*cos(q4)*sin(q5) - 0.0053163*dq2*cos(q2)*cos(q5)*sin(q4) - 2.0e-9*dq3*cos(q2)*cos(q3)*sin(q5) + 0.00024178*dq3*cos(q2)*cos(q5)*sin(q3) - 0.00024178*dq3*cos(q3)*cos(q5)*sin(q2) - 0.0010941*dq4*cos(q2)*cos(q4)*sin(q3) + 0.0010941*dq4*cos(q3)*cos(q4)*sin(q2) - 0.00024178*dq4*cos(q2)*cos(q3)*sin(q5) - 6.0e-8*dq4*cos(q4)*cos(q5)*sin(q2) + 1.3553e-20*dq5*cos(q2)*cos(q3)*sin(q5) - 5.0e-9*dq5*cos(q2)*cos(q5)*sin(q3) + 5.0e-9*dq5*cos(q3)*cos(q5)*sin(q2) - 4.0e-8*dq5*cos(q4)*cos(q5)*sin(q2) + 0.000234*dq6*cos(q2)*cos(q3)*sin(q5) + 0.0010941*dq2*sin(q2)*sin(q3)*sin(q4) + 2.0e-9*dq2*sin(q2)*sin(q3)*sin(q5) - 0.0010941*dq3*sin(q2)*sin(q3)*sin(q4) - 0.0013291*dq1*sin(q3)*sin(q4)*sin(q5) - 2.0e-9*dq3*sin(q2)*sin(q3)*sin(q5) - 0.00024178*dq4*sin(q2)*sin(q3)*sin(q5) + 4.0e-8*dq4*sin(q2)*sin(q4)*sin(q5) + 1.3553e-20*dq5*sin(q2)*sin(q3)*sin(q5) + 6.0e-8*dq5*sin(q2)*sin(q4)*sin(q5) + 0.000234*dq6*sin(q2)*sin(q3)*sin(q5) - 0.0014978*dq1*cos(2.0*q2)*cos(2.0*q3)*sin(q5) - 0.0014978*dq1*sin(2.0*q2)*sin(2.0*q3)*sin(q5) + 0.002302*dq1*cos(2.0*q2)*cos(q3)*sin(q5) - 0.00065996*dq4*sin(2.0*q5)*cos(q2)*cos(q3) + 0.000060445*dq1*cos(2.0*q2)*cos(2.0*q3)*cos(2.0*q4)*sin(q5) + 0.00012089*dq1*cos(2.0*q2)*cos(2.0*q3)*sin(2.0*q4)*cos(q5) + 0.00076206*dq1*cos(2.0*q2)*cos(2.0*q5)*sin(2.0*q3)*cos(q4) - 0.00076206*dq1*cos(2.0*q3)*cos(2.0*q5)*sin(2.0*q2)*cos(q4) - 0.00038102*dq1*cos(2.0*q2)*sin(2.0*q3)*sin(2.0*q5)*sin(q4) + 0.00038102*dq1*cos(2.0*q3)*sin(2.0*q2)*sin(2.0*q5)*sin(q4) + 0.000060445*dq1*cos(2.0*q4)*sin(2.0*q2)*sin(2.0*q3)*sin(q5) + 0.00012089*dq1*sin(2.0*q2)*sin(2.0*q3)*sin(2.0*q4)*cos(q5) + 0.0016597*dq2*cos(q2)*cos(q3)*cos(q4)*sin(q5) + 0.0033194*dq2*cos(q2)*cos(q3)*cos(q5)*sin(q4) - 3.0e-8*dq2*cos(q2)*cos(q4)*cos(q5)*sin(q3) + 3.0e-8*dq2*cos(q3)*cos(q4)*cos(q5)*sin(q2) - 0.0016597*dq3*cos(q2)*cos(q3)*cos(q4)*sin(q5) - 0.0033194*dq3*cos(q2)*cos(q3)*cos(q5)*sin(q4) + 3.0e-8*dq3*cos(q2)*cos(q4)*cos(q5)*sin(q3) - 3.0e-8*dq3*cos(q3)*cos(q4)*cos(q5)*sin(q2) + 2.35e-8*dq4*cos(q2)*cos(q3)*cos(q4)*sin(q5) + 3.0e-8*dq4*cos(q2)*cos(q3)*cos(q5)*sin(q4) - 3.5e-8*dq4*cos(q2)*cos(q4)*cos(q5)*sin(q3) + 3.5e-8*dq4*cos(q3)*cos(q4)*cos(q5)*sin(q2) + 2.5e-8*dq5*cos(q2)*cos(q3)*cos(q4)*sin(q5) + 2.85e-8*dq5*cos(q2)*cos(q3)*cos(q5)*sin(q4) - 3.0e-8*dq5*cos(q2)*cos(q4)*cos(q5)*sin(q3) + 3.0e-8*dq5*cos(q3)*cos(q4)*cos(q5)*sin(q2) - 0.0002702*dq6*cos(q2)*cos(q4)*cos(q5)*sin(q3) + 0.0002702*dq6*cos(q3)*cos(q4)*cos(q5)*sin(q2) + 2.35e-8*dq2*cos(q2)*sin(q3)*sin(q4)*sin(q5) - 2.35e-8*dq2*cos(q3)*sin(q2)*sin(q4)*sin(q5) + 0.0016597*dq2*cos(q4)*sin(q2)*sin(q3)*sin(q5) + 0.0033194*dq2*cos(q5)*sin(q2)*sin(q3)*sin(q4) - 2.35e-8*dq3*cos(q2)*sin(q3)*sin(q4)*sin(q5) + 2.35e-8*dq3*cos(q3)*sin(q2)*sin(q4)*sin(q5) - 0.0016597*dq3*cos(q4)*sin(q2)*sin(q3)*sin(q5) - 0.0033194*dq3*cos(q5)*sin(q2)*sin(q3)*sin(q4) + 0.00041882*dq4*cos(q2)*sin(q3)*sin(q4)*sin(q5) - 0.00041882*dq4*cos(q3)*sin(q2)*sin(q4)*sin(q5) + 2.35e-8*dq4*cos(q4)*sin(q2)*sin(q3)*sin(q5) + 3.0e-8*dq4*cos(q5)*sin(q2)*sin(q3)*sin(q4) + 2.0e-8*dq5*cos(q2)*sin(q3)*sin(q4)*sin(q5) - 2.0e-8*dq5*cos(q3)*sin(q2)*sin(q4)*sin(q5) + 2.5e-8*dq5*cos(q4)*sin(q2)*sin(q3)*sin(q5) + 2.85e-8*dq5*cos(q5)*sin(q2)*sin(q3)*sin(q4) + 0.0001351*dq6*cos(q2)*sin(q3)*sin(q4)*sin(q5) - 0.0001351*dq6*cos(q3)*sin(q2)*sin(q4)*sin(q5) + 0.0016597*dq1*cos(2.0*q2)*sin(2.0*q3)*cos(q4)*cos(q5) - 0.0016597*dq1*cos(2.0*q3)*sin(2.0*q2)*cos(q4)*cos(q5) - 0.00043998*dq2*cos(2.0*q4)*cos(2.0*q5)*cos(q2)*sin(q3) + 0.00043998*dq2*cos(2.0*q4)*cos(2.0*q5)*cos(q3)*sin(q2) + 0.00043998*dq3*cos(2.0*q4)*cos(2.0*q5)*cos(q2)*sin(q3) - 0.00043998*dq3*cos(2.0*q4)*cos(2.0*q5)*cos(q3)*sin(q2) - 0.00062049*dq1*cos(2.0*q2)*sin(2.0*q3)*sin(q4)*sin(q5) + 0.00062049*dq1*cos(2.0*q3)*sin(2.0*q2)*sin(q4)*sin(q5) + 0.00054998*dq2*sin(2.0*q4)*sin(2.0*q5)*cos(q2)*sin(q3) - 0.00054998*dq2*sin(2.0*q4)*sin(2.0*q5)*cos(q3)*sin(q2) - 0.00054998*dq3*sin(2.0*q4)*sin(2.0*q5)*cos(q2)*sin(q3) + 0.00054998*dq3*sin(2.0*q4)*sin(2.0*q5)*cos(q3)*sin(q2) - 0.00027498*dq1*cos(2.0*q2)*cos(2.0*q3)*cos(2.0*q4)*sin(2.0*q5) - 0.00021998*dq1*cos(2.0*q2)*cos(2.0*q3)*cos(2.0*q5)*sin(2.0*q4) - 0.00027498*dq1*cos(2.0*q4)*sin(2.0*q2)*sin(2.0*q3)*sin(2.0*q5) - 0.00021998*dq1*cos(2.0*q5)*sin(2.0*q2)*sin(2.0*q3)*sin(2.0*q4) - 0.0026581*dq1*cos(2.0*q2)*cos(q4)*cos(q5)*sin(q3) + 0.0026581*dq1*sin(2.0*q2)*cos(q3)*cos(q4)*cos(q5) + 0.00024178*dq2*cos(2.0*q4)*cos(q2)*cos(q5)*sin(q3) - 0.00024178*dq2*cos(2.0*q4)*cos(q3)*cos(q5)*sin(q2) + 0.00076206*dq2*cos(2.0*q5)*cos(q2)*cos(q3)*sin(q4) + 0.00038102*dq2*sin(2.0*q5)*cos(q2)*cos(q3)*cos(q4) - 0.00024178*dq3*cos(2.0*q4)*cos(q2)*cos(q5)*sin(q3) + 0.00024178*dq3*cos(2.0*q4)*cos(q3)*cos(q5)*sin(q2) - 0.00076206*dq3*cos(2.0*q5)*cos(q2)*cos(q3)*sin(q4) - 0.00038102*dq3*sin(2.0*q5)*cos(q2)*cos(q3)*cos(q4) + 0.00076206*dq4*cos(2.0*q5)*cos(q2)*cos(q4)*sin(q3) - 0.00076206*dq4*cos(2.0*q5)*cos(q3)*cos(q4)*sin(q2) + 0.0013291*dq1*cos(2.0*q2)*sin(q3)*sin(q4)*sin(q5) - 0.0013291*dq1*sin(2.0*q2)*cos(q3)*sin(q4)*sin(q5) + 0.00076206*dq2*cos(2.0*q5)*sin(q2)*sin(q3)*sin(q4) - 0.00012089*dq2*sin(2.0*q4)*cos(q2)*sin(q3)*sin(q5) + 0.00012089*dq2*sin(2.0*q4)*cos(q3)*sin(q2)*sin(q5) + 0.00038102*dq2*sin(2.0*q5)*cos(q4)*sin(q2)*sin(q3) - 0.00076206*dq3*cos(2.0*q5)*sin(q2)*sin(q3)*sin(q4) + 0.00012089*dq3*sin(2.0*q4)*cos(q2)*sin(q3)*sin(q5) - 0.00012089*dq3*sin(2.0*q4)*cos(q3)*sin(q2)*sin(q5) - 0.00038102*dq3*sin(2.0*q5)*cos(q4)*sin(q2)*sin(q3) - 0.00038102*dq4*sin(2.0*q5)*cos(q2)*sin(q3)*sin(q4) + 0.00038102*dq4*sin(2.0*q5)*cos(q3)*sin(q2)*sin(q4);
 
C5_2 = 0.00032998*dq2*sin(2.0*q5) - 0.00032998*dq3*sin(2.0*q5) + 0.0027538*dq2*sin(q5) - 0.0027538*dq3*sin(q5) - 0.0010941*dq4*sin(q4) - 0.5*dq6*(0.0002702*cos(q4)*sin(q5) + 0.0005404*cos(q5)*sin(q4)) + 0.00012089*dq2*cos(2.0*q4)*sin(q5) + 0.00024178*dq2*sin(2.0*q4)*cos(q5) - 0.00012089*dq3*cos(2.0*q4)*sin(q5) - 0.00024178*dq3*sin(2.0*q4)*cos(q5) + 0.00076206*dq4*cos(2.0*q5)*sin(q4) + 0.00038103*dq4*sin(2.0*q5)*cos(q4) + 0.0006317*dq1*cos(q2)*sin(q3) - 0.0006317*dq1*cos(q3)*sin(q2) - 0.0046041*dq2*cos(q3)*sin(q5) - 0.0004188*dq4*cos(q4)*sin(q5) - 0.00054997*dq2*cos(2.0*q4)*sin(2.0*q5) - 0.00043998*dq2*cos(2.0*q5)*sin(2.0*q4) + 0.00054997*dq3*cos(2.0*q4)*sin(2.0*q5) + 0.00043998*dq3*cos(2.0*q5)*sin(2.0*q4) + 0.0010941*dq1*cos(q2)*cos(q3)*sin(q4) - 0.00024178*dq1*cos(q2)*cos(q5)*sin(q3) + 0.00024178*dq1*cos(q3)*cos(q5)*sin(q2) - 0.0026582*dq1*cos(q2)*cos(q4)*sin(q5) - 0.0053164*dq1*cos(q2)*cos(q5)*sin(q4) + 0.0053165*dq2*cos(q4)*cos(q5)*sin(q3) + 0.0010941*dq1*sin(q2)*sin(q3)*sin(q4) - 0.0026582*dq2*sin(q3)*sin(q4)*sin(q5) + 0.0016597*dq1*cos(q2)*cos(q3)*cos(q4)*sin(q5) + 0.0033194*dq1*cos(q2)*cos(q3)*cos(q5)*sin(q4) + 0.0016597*dq1*cos(q4)*sin(q2)*sin(q3)*sin(q5) + 0.0033194*dq1*cos(q5)*sin(q2)*sin(q3)*sin(q4) - 0.00043998*dq1*cos(2.0*q4)*cos(2.0*q5)*cos(q2)*sin(q3) + 0.00043998*dq1*cos(2.0*q4)*cos(2.0*q5)*cos(q3)*sin(q2) + 0.00054997*dq1*sin(2.0*q4)*sin(2.0*q5)*cos(q2)*sin(q3) - 0.00054997*dq1*sin(2.0*q4)*sin(2.0*q5)*cos(q3)*sin(q2) + 0.00024178*dq1*cos(2.0*q4)*cos(q2)*cos(q5)*sin(q3) - 0.00024178*dq1*cos(2.0*q4)*cos(q3)*cos(q5)*sin(q2) + 0.00076206*dq1*cos(2.0*q5)*cos(q2)*cos(q3)*sin(q4) + 0.00038103*dq1*sin(2.0*q5)*cos(q2)*cos(q3)*cos(q4) + 0.00076206*dq1*cos(2.0*q5)*sin(q2)*sin(q3)*sin(q4) - 0.00012089*dq1*sin(2.0*q4)*cos(q2)*sin(q3)*sin(q5) + 0.00012089*dq1*sin(2.0*q4)*cos(q3)*sin(q2)*sin(q5) + 0.00038103*dq1*sin(2.0*q5)*cos(q4)*sin(q2)*sin(q3);
 
C5_3 = 0.00032998*dq3*sin(2.0*q5) - 0.00032998*dq2*sin(2.0*q5) - 0.0027538*dq2*sin(q5) + 0.0027538*dq3*sin(q5) + 0.0010941*dq4*sin(q4) - 0.00012089*dq2*cos(2.0*q4)*sin(q5) - 0.00024178*dq2*sin(2.0*q4)*cos(q5) + 0.00012089*dq3*cos(2.0*q4)*sin(q5) + 0.00024178*dq3*sin(2.0*q4)*cos(q5) - 0.00076206*dq4*cos(2.0*q5)*sin(q4) - 0.00038103*dq4*sin(2.0*q5)*cos(q4) - 0.0006317*dq1*cos(q2)*sin(q3) + 0.0006317*dq1*cos(q3)*sin(q2) + 0.0004188*dq4*cos(q4)*sin(q5) + 0.0001351*dq6*cos(q4)*sin(q5) + 0.0002702*dq6*cos(q5)*sin(q4) + 0.00054997*dq2*cos(2.0*q4)*sin(2.0*q5) + 0.00043998*dq2*cos(2.0*q5)*sin(2.0*q4) - 0.00054997*dq3*cos(2.0*q4)*sin(2.0*q5) - 0.00043998*dq3*cos(2.0*q5)*sin(2.0*q4) - 0.0010941*dq1*cos(q2)*cos(q3)*sin(q4) + 0.00024178*dq1*cos(q2)*cos(q5)*sin(q3) - 0.00024178*dq1*cos(q3)*cos(q5)*sin(q2) - 0.0010941*dq1*sin(q2)*sin(q3)*sin(q4) - 0.0016597*dq1*cos(q2)*cos(q3)*cos(q4)*sin(q5) - 0.0033194*dq1*cos(q2)*cos(q3)*cos(q5)*sin(q4) - 0.0016597*dq1*cos(q4)*sin(q2)*sin(q3)*sin(q5) - 0.0033194*dq1*cos(q5)*sin(q2)*sin(q3)*sin(q4) + 0.00043998*dq1*cos(2.0*q4)*cos(2.0*q5)*cos(q2)*sin(q3) - 0.00043998*dq1*cos(2.0*q4)*cos(2.0*q5)*cos(q3)*sin(q2) - 0.00054997*dq1*sin(2.0*q4)*sin(2.0*q5)*cos(q2)*sin(q3) + 0.00054997*dq1*sin(2.0*q4)*sin(2.0*q5)*cos(q3)*sin(q2) - 0.00024178*dq1*cos(2.0*q4)*cos(q2)*cos(q5)*sin(q3) + 0.00024178*dq1*cos(2.0*q4)*cos(q3)*cos(q5)*sin(q2) - 0.00076206*dq1*cos(2.0*q5)*cos(q2)*cos(q3)*sin(q4) - 0.00038103*dq1*sin(2.0*q5)*cos(q2)*cos(q3)*cos(q4) - 0.00076206*dq1*cos(2.0*q5)*sin(q2)*sin(q3)*sin(q4) + 0.00012089*dq1*sin(2.0*q4)*cos(q2)*sin(q3)*sin(q5) - 0.00012089*dq1*sin(2.0*q4)*cos(q3)*sin(q2)*sin(q5) - 0.00038103*dq1*sin(2.0*q5)*cos(q4)*sin(q2)*sin(q3);
 
C5_4 = 0.0018562*dq3*sin(q4) - 0.0018562*dq2*sin(q4) - 0.5*dq4*(0.0013199*sin(2.0*q5) + 0.00048356*sin(q5)) + 0.000234*dq6*sin(q5) - 0.0004188*dq2*cos(q4)*sin(q5) + 0.0004188*dq3*cos(q4)*sin(q5) + 0.0015241*dq2*cos(q5)^2*sin(q4) - 0.0015241*dq3*cos(q5)^2*sin(q4) - 0.0018562*dq1*cos(q2)*cos(q4)*sin(q3) + 0.0018562*dq1*cos(q3)*cos(q4)*sin(q2) - 0.00024178*dq1*cos(q2)*cos(q3)*sin(q5) + 0.00076206*dq2*cos(q4)*cos(q5)*sin(q5) - 0.00076206*dq3*cos(q4)*cos(q5)*sin(q5) - 0.00024178*dq1*sin(q2)*sin(q3)*sin(q5) - 0.0013199*dq1*cos(q2)*cos(q3)*cos(q5)*sin(q5) + 0.0004188*dq1*cos(q2)*sin(q3)*sin(q4)*sin(q5) - 0.0004188*dq1*cos(q3)*sin(q2)*sin(q4)*sin(q5) - 0.0013199*dq1*cos(q5)*sin(q2)*sin(q3)*sin(q5) + 0.0015241*dq1*cos(q2)*cos(q4)*cos(q5)^2*sin(q3) - 0.0015241*dq1*cos(q3)*cos(q4)*cos(q5)^2*sin(q2) - 0.00076206*dq1*cos(q2)*cos(q5)*sin(q3)*sin(q4)*sin(q5) + 0.00076206*dq1*cos(q3)*cos(q5)*sin(q2)*sin(q4)*sin(q5);
 
C5_5 = 0.0;
 
C5_6 = 0.5*dq1*(0.000468*cos(q2 - 1.0*q3)*sin(q5) + 0.0005404*sin(q2 - 1.0*q3)*cos(q4)*cos(q5) - 0.0002702*sin(q2 - 1.0*q3)*sin(q4)*sin(q5)) + 0.000234*dq4*sin(q5) - 0.5*dq2*(0.0002702*cos(q4)*sin(q5) + 0.0005404*cos(q5)*sin(q4)) + 0.5*dq3*(0.0002702*cos(q4)*sin(q5) + 0.0005404*cos(q5)*sin(q4));
 
C6_1 = 0.0001351*cos(q2 - 1.0*q3)*sin(q4)*(dq2 - 1.0*dq3) - 0.000078*sin(q2 - 1.0*q3)*(dq2 - 1.0*dq3) - 0.000234*sin(q2 - 1.0*q3)*cos(q5)*(dq2 - 1.0*dq3) + 0.0001351*dq4*sin(q2 - 1.0*q3)*cos(q4) - 0.000234*dq5*cos(q2 - 1.0*q3)*sin(q5) - 0.0002702*cos(q2 - 1.0*q3)*cos(q4)*sin(q5)*(dq2 - 1.0*dq3) - 0.0001351*cos(q2 - 1.0*q3)*cos(q5)*sin(q4)*(dq2 - 1.0*dq3) - 0.0001351*dq4*sin(q2 - 1.0*q3)*cos(q4)*cos(q5) - 0.0002702*dq5*sin(q2 - 1.0*q3)*cos(q4)*cos(q5) + 0.0002702*dq4*sin(q2 - 1.0*q3)*sin(q4)*sin(q5) + 0.0001351*dq5*sin(q2 - 1.0*q3)*sin(q4)*sin(q5);
 
C6_2 = 0.0002702*dq4*cos(q4)*sin(q5) - 0.0001351*dq4*sin(q4) - 0.000078*dq1*sin(q2 - 1.0*q3) + 0.0001351*dq4*cos(q5)*sin(q4) + 0.0001351*dq5*cos(q4)*sin(q5) + 0.0002702*dq5*cos(q5)*sin(q4) + 0.0001351*dq1*cos(q2 - 1.0*q3)*sin(q4) - 0.000234*dq1*sin(q2 - 1.0*q3)*cos(q5) - 0.0002702*dq1*cos(q2 - 1.0*q3)*cos(q4)*sin(q5) - 0.0001351*dq1*cos(q2 - 1.0*q3)*cos(q5)*sin(q4); 

C6_3 = 0.000078*dq1*sin(q2 - 1.0*q3) + 0.0001351*dq4*sin(q4) - 0.0002702*dq4*cos(q4)*sin(q5) - 0.0001351*dq4*cos(q5)*sin(q4) - 0.0001351*dq5*cos(q4)*sin(q5) - 0.0002702*dq5*cos(q5)*sin(q4) - 0.0001351*dq1*cos(q2 - 1.0*q3)*sin(q4) + 0.000234*dq1*sin(q2 - 1.0*q3)*cos(q5) + 0.0002702*dq1*cos(q2 - 1.0*q3)*cos(q4)*sin(q5) + 0.0001351*dq1*cos(q2 - 1.0*q3)*cos(q5)*sin(q4);
 
C6_4 = 0.0001351*dq2*(2.0*cos(q4)*sin(q5) - 1.0*sin(q4) + cos(q5)*sin(q4)) - 0.0001351*dq3*(2.0*cos(q4)*sin(q5) - 1.0*sin(q4) + cos(q5)*sin(q4)) - 0.000234*dq5*sin(q5) + 0.0001351*dq1*sin(q2 - 1.0*q3)*(cos(q4) - 1.0*cos(q4)*cos(q5) + 2.0*sin(q4)*sin(q5));
 
C6_5 = 0.5*dq2*(0.0002702*cos(q4)*sin(q5) + 0.0005404*cos(q5)*sin(q4)) - 0.000234*dq4*sin(q5) - 0.5*dq1*(0.000468*cos(q2 - 1.0*q3)*sin(q5) + 0.0005404*sin(q2 - 1.0*q3)*cos(q4)*cos(q5) - 0.0002702*sin(q2 - 1.0*q3)*sin(q4)*sin(q5)) - 0.5*dq3*(0.0002702*cos(q4)*sin(q5) + 0.0005404*cos(q5)*sin(q4));
 
C6_6 = 0.0; 
 
C =[C1_1, C1_2, C1_3, C1_4, C1_5, C1_6;
    C2_1, C2_2, C2_3, C2_4, C2_5, C2_6;
    C3_1, C3_2, C3_3, C3_4, C3_5, C3_6;
    C4_1, C4_2, C4_3, C4_4, C4_5, C4_6;
    C5_1, C5_2, C5_3, C5_4, C5_5, C5_6;
    C6_1, C6_2, C6_3, C6_4, C6_5, C6_6];
